simulink model "simulator_prototype_v2"  (R2021b)
settings: Solver=VariableStepAuto  StartTime=0.0  StopTime=60  FixedStep=0.0001  RelTol=1e-4
values from neighbouring files (symbols this model uses):
  N = length(mass)    [inertia_matrix.m]
undefined symbols (not defined in the file or in its folder): X, Y, Z
libraries: sm_lib x47, nesl_utility x7
(part 4 of 12)

== matlab function simulator_prototype_v2/Dynamic Model/Coriolis_vector_v2 ==
  data: dq1 input; tau_c output; dq2 input; dq3 input; dq4 input; dq5 input; dq6 input; q1 input; q2 input; q3 input; q4 input; q5 input; q6 input
function tau_c = Coriolis_vector_v2(dq1,dq2,dq3,dq4,dq5,dq6,q1,q2,q3,q4,q5,q6)
%#codegen

%    This function was generated by the Symbolic Math Toolbox version 9.0.
%    06-Nov-2021 23:01:03

t2 = conj(dq1);
t3 = conj(dq2);
t4 = conj(dq3);
t5 = conj(dq4);
t6 = conj(dq5);
t7 = conj(dq6);
t8 = conj(q1);
t9 = conj(q2);
t10 = conj(q3);
t11 = conj(q4);
t12 = conj(q5);
t13 = conj(q6);
t14 = cos(q1);
t15 = cos(q2);
t16 = cos(q4);
t17 = cos(q5);
t18 = cos(q6);
t19 = sin(q1);
t20 = sin(q2);
t21 = sin(q4);
t22 = sin(q5);
t23 = sin(q6);
t29 = q1+q2;
t50 = 9.007199254740992e+15;
t24 = cos(t8);
t25 = cos(t9);
t26 = cos(t11);
t27 = cos(t12);
t28 = cos(t13);
t30 = sin(t8);
t31 = sin(t9);
t32 = sin(t11);
t33 = sin(t12);
t34 = sin(t13);
t35 = cos(t29);
t36 = sin(t29);
t37 = t8+t9;
t51 = t17.*3.347317932164228e+33;
t52 = t22.*3.347317932164228e+33;
t56 = t14.*4.990478e-2;
t58 = t19.*4.990478e-2;
t59 = t14.*2.167433e-2;
t60 = t19.*2.167433e-2;
t61 = t16.*t18.*3.315051378778914e+33;
t62 = t14.*t15.*3.641522e-2;
t63 = t16.*t23.*3.315051378778914e+33;
t64 = t18.*t21.*3.315051378778914e+33;
t65 = t16.*t22.*1.990083581481952e+33;
t66 = t17.*t21.*1.990083581481952e+33;
t67 = t14.*t20.*3.641522e-2;
t68 = t15.*t19.*3.641522e-2;
t69 = t21.*t22.*1.990083581481952e+33;
t70 = t19.*t20.*3.641522e-2;
t74 = t19.*t20.*2.462267e-2;
t78 = t17.*t18.*5.575912001630188e+33;
t79 = t16.*t18.*6.099194893302011e+33;
t80 = t17.*t18.*1.025883768304404e+34;
t81 = t17.*t23.*5.575912001630188e+33;
t82 = t16.*t23.*6.099194893302011e+33;
t83 = t17.*t23.*1.025883768304404e+34;
t84 = t18.*t22.*1.025883768304404e+34;
t85 = t22.*t23.*5.575912001630188e+33;
t87 = t21.*t23.*6.099194893302011e+33;
t89 = t14.*t15.*2.462267e-2;
t90 = t14.*t20.*2.462267e-2;
t91 = t15.*t19.*2.462267e-2;
t93 = t21.*t22.*t23.*3.315051378778914e+33;
t105 = t17.*t21.*t23.*3.315051378778914e+33;
t116 = t17.*t18.*t21.*6.099194893302011e+33;
t118 = t18.*t21.*t22.*6.099194893302011e+33;
t127 = t21.*t22.*t23.*-6.099194893302011e+33;
t142 = t16.*7.746286054220548e+49;
t143 = t21.*7.746286054220548e+49;
t144 = t16.*t22.*1.830618490855195e+48;
t145 = t17.*t21.*1.830618490855195e+48;
t150 = t16.*t17.*1.830618490855195e+48;
t153 = t16.*t17.*7.290917220067534e+49;
t154 = t16.*t22.*7.290917220067534e+49;
t155 = t21.*t22.*7.290917220067534e+49;
t158 = t16.*6.997781708721691e+52;
t159 = t21.*6.997781708721691e+52;
t166 = t16.*t17.*t18.*5.84291401185902e+49;
t168 = t16.*t17.*t23.*5.84291401185902e+49;
t170 = t16.*t22.*t23.*5.84291401185902e+49;
t171 = t17.*t21.*t23.*5.84291401185902e+49;
t174 = t16.*t22.*7.183572847808854e+52;
t175 = t17.*t21.*7.183572847808854e+52;
t177 = t21.*t22.*7.183572847808854e+52;
t178 = t16.*t17.*t18.*1.075008113939401e+50;
t179 = t16.*t17.*t23.*1.075008113939401e+50;
t180 = t16.*t18.*t22.*1.075008113939401e+50;
t181 = t17.*t18.*t21.*1.075008113939401e+50;
t183 = (q3.*t50)./9.007199254740992e+15;
t184 = t16.*t18.*1.196628789628727e+53;
t185 = t16.*t23.*1.196628789628727e+53;
t186 = t18.*t21.*1.196628789628727e+53;
t187 = (t10.*t50)./9.007199254740992e+15;
t191 = t16.*t18.*2.201616617347892e+53;
t192 = t16.*t23.*2.201616617347892e+53;
t193 = q3.*t50.*2.220446049250313e-16i;
t194 = t21.*t23.*2.201616617347892e+53;
t199 = t10.*t50.*2.220446049250313e-16i;
t206 = q3.*t50.*1.110223024625157e-16i;
t210 = t17.*t21.*t23.*1.196628789628727e+53;
t212 = t21.*t22.*t23.*1.196628789628727e+53;
t214 = t10.*t50.*1.110223024625157e-16i;
t219 = t17.*t18.*t21.*2.201616617347892e+53;
t221 = t18.*t21.*t22.*2.201616617347892e+53;
t232 = t16.*t17.*t50.*4.323455642275676e+17i;
t233 = t16.*t22.*t50.*4.323455642275676e+17i;
t234 = t21.*t22.*t50.*4.323455642275676e+17i;
t242 = t21.*t22.*t23.*-2.201616617347892e+53;
t247 = t16.*t18.*t50.*7.201947557068188e+17i;
t248 = t16.*t23.*t50.*1.325049802940888e+18i;
t249 = t18.*t21.*t50.*1.325049802940888e+18i;
t251 = t18.*t21.*t50.*7.201947557068188e+17i;
t253 = t21.*t23.*t50.*1.325049802940888e+18i;
t254 = t21.*t23.*t50.*7.201947557068188e+17i;
t278 = t16.*t17.*t18.*t50.*1.325049802940888e+18i;
t282 = t16.*t18.*t22.*t50.*1.325049802940888e+18i;
t284 = t16.*t17.*t23.*t50.*7.201947557068188e+17i;
t289 = t16.*t22.*t23.*t50.*7.201947557068188e+17i;
t297 = t16.*t22.*t23.*t50.*-1.325049802940888e+18i;
t298 = t18.*t21.*t22.*t50.*-1.325049802940888e+18i;
t299 = t21.*t22.*t23.*t50.*-7.201947557068188e+17i;
t353 = t17.*t50.*1.746965228796509e+32i;
t355 = t22.*t50.*1.746965228796509e+32i;
t375 = t16.*t50.*4.394953650240249e+33i;
t377 = t21.*t50.*4.394953650240249e+33i;
t379 = t17.*t21.*t50.*1.03862462117543e+32i;
t383 = t21.*t22.*t50.*1.03862462117543e+32i;
t385 = t17.*t50.*6.957746211523004e+33i;
t386 = t22.*t50.*6.957746211523004e+33i;
t390 = t16.*t17.*t50.*1.03862462117543e+32i;
t394 = t16.*t22.*t50.*4.136594366080324e+33i;
t395 = t17.*t21.*t50.*4.136594366080324e+33i;
t396 = t21.*t22.*t50.*4.136594366080324e+33i;
t399 = t16.*t50.*3.97028021545552e+36i;
t400 = t21.*t50.*3.97028021545552e+36i;
t401 = t17.*t18.*t50.*1.025883768304404e+34i;
t402 = t17.*t23.*t50.*5.575912001630188e+33i;
t403 = t18.*t22.*t50.*5.575912001630188e+33i;
t404 = t18.*t22.*t50.*1.025883768304404e+34i;
t406 = t22.*t23.*t50.*5.575912001630188e+33i;
t409 = t22.*t23.*t50.*1.025883768304404e+34i;
t415 = t16.*t17.*t23.*t50.*3.315051378778914e+33i;
t416 = t17.*t18.*t21.*t50.*3.315051378778914e+33i;
t417 = t17.*t21.*t23.*t50.*3.315051378778914e+33i;
t418 = t21.*t22.*t23.*t50.*3.315051378778914e+33i;
t433 = t16.*t17.*t50.*4.075691174875038e+36i;
t435 = t16.*t22.*t50.*4.075691174875038e+36i;
t436 = t21.*t22.*t50.*4.075691174875038e+36i;
t440 = t16.*t17.*t18.*t50.*6.099194893302011e+33i;
t443 = t17.*t18.*t21.*t50.*6.099194893302011e+33i;
t446 = t17.*t21.*t23.*t50.*6.099194893302011e+33i;
t447 = t18.*t21.*t22.*t50.*6.099194893302011e+33i;
t448 = t16.*t18.*t50.*6.789225223739216e+36i;
t449 = t16.*t23.*t50.*1.249115114148252e+37i;
t450 = t18.*t21.*t50.*1.249115114148252e+37i;
t451 = t18.*t21.*t50.*6.789225223739216e+36i;
t453 = t21.*t23.*t50.*1.249115114148252e+37i;
t454 = t21.*t23.*t50.*6.789225223739216e+36i;
t472 = t16.*t17.*t18.*t50.*1.249115114148252e+37i;
t476 = t16.*t18.*t22.*t50.*1.249115114148252e+37i;
t477 = t16.*t17.*t23.*t50.*6.789225223739216e+36i;
t483 = t16.*t22.*t23.*t50.*6.789225223739216e+36i;
t494 = t16.*t22.*t23.*t50.*-1.249115114148252e+37i;
t495 = t18.*t21.*t22.*t50.*-1.249115114148252e+37i;
t496 = t21.*t22.*t23.*t50.*-6.789225223739216e+36i;
t583 = t14.*t15.*3.15365435562893e-2;
t584 = t14.*t20.*3.15365435562893e-2;
t585 = t15.*t19.*3.15365435562893e-2;
t586 = t14.*t15.*2.561099610858757e-2;
t588 = t19.*t20.*3.15365435562893e-2;
t589 = t14.*t20.*2.561099610858757e-2;
t590 = t15.*t19.*2.561099610858757e-2;
t592 = t19.*t20.*2.561099610858757e-2;
t597 = t14.*t15.*1.57299335562893e-2;
t600 = t14.*t20.*1.57299335562893e-2;
t601 = t15.*t19.*1.57299335562893e-2;
t603 = t19.*t20.*1.57299335562893e-2;
t604 = t14.*t15.*4.804434610858757e-2;
t605 = t14.*t20.*4.804434610858757e-2;
t606 = t15.*t19.*4.804434610858757e-2;
t607 = t19.*t20.*4.804434610858757e-2;
t626 = t14.*t15.*1.919581841189621e-2;
t628 = t14.*t15.*4.735389991350965e-2;
t632 = t14.*t20.*1.919581841189621e-2;
t633 = t15.*t19.*1.919581841189621e-2;
t635 = t14.*t20.*4.735389991350965e-2;
t636 = t15.*t19.*4.735389991350965e-2;
t638 = t19.*t20.*1.919581841189621e-2;
t639 = t19.*t20.*4.735389991350965e-2;
t640 = t14.*t15.*2.273122991350965e-2;
t641 = t14.*t15.*3.603517512464e-2;
t642 = t14.*t20.*2.273122991350965e-2;
t643 = t15.*t19.*2.273122991350965e-2;
t645 = t14.*t20.*3.603517512464e-2;
t646 = t15.*t19.*3.603517512464e-2;
t647 = t19.*t20.*2.273122991350965e-2;
t649 = t19.*t20.*3.603517512464e-2;
t653 = t14.*t15.*1.141250512464e-2;
t654 = t14.*t20.*1.141250512464e-2;
t655 = t15.*t19.*1.141250512464e-2;
t656 = t19.*t20.*1.141250512464e-2;
t661 = t14.*t15.*5.561103841189621e-2;
t663 = t14.*t20.*5.561103841189621e-2;
t664 = t15.*t19.*5.561103841189621e-2;
t666 = t19.*t20.*5.561103841189621e-2;
t667 = t14.*t15.*3.823389842399381e-2;
t668 = t14.*t20.*3.823389842399381e-2;
t669 = t15.*t19.*3.823389842399381e-2;
t671 = t14.*t15.*7.464911842399381e-2;
t674 = t19.*t20.*3.823389842399381e-2;
t675 = t14.*t20.*7.464911842399381e-2;
t676 = t15.*t19.*7.464911842399381e-2;
t679 = t19.*t20.*7.464911842399381e-2;
t703 = t14.*t15.*t16.*t22.*2.498039274760989e-3;
t704 = t14.*t16.*t17.*t20.*2.498039274760989e-3;
t705 = t15.*t16.*t17.*t19.*2.498039274760989e-3;
t706 = t14.*t15.*t21.*t22.*2.498039274760989e-3;
t707 = t14.*t16.*t20.*t22.*2.498039274760989e-3;
t708 = t15.*t16.*t19.*t22.*2.498039274760989e-3;
t709 = t16.*t17.*t19.*t20.*2.498039274760989e-3;
t711 = t14.*t15.*t16.*t17.*5.478347731418506e-3;
t712 = t14.*t20.*t21.*t22.*2.498039274760989e-3;
t713 = t15.*t19.*t21.*t22.*2.498039274760989e-3;
t714 = t16.*t19.*t20.*t22.*2.498039274760989e-3;
t719 = t14.*t15.*t16.*t22.*5.478347731418506e-3;
t720 = t14.*t15.*t17.*t21.*5.478347731418506e-3;
t721 = t14.*t16.*t17.*t20.*5.478347731418506e-3;
t722 = t15.*t16.*t17.*t19.*5.478347731418506e-3;
t723 = t19.*t20.*t21.*t22.*2.498039274760989e-3;
t726 = t14.*t16.*t20.*t22.*5.478347731418506e-3;
t727 = t14.*t17.*t20.*t21.*5.478347731418506e-3;
t728 = t15.*t16.*t19.*t22.*5.478347731418506e-3;
t729 = t15.*t17.*t19.*t21.*5.478347731418506e-3;
t730 = t16.*t17.*t19.*t20.*5.478347731418506e-3;
t731 = t16.*t19.*t20.*t22.*5.478347731418506e-3;
t732 = t17.*t19.*t20.*t21.*5.478347731418506e-3;
t742 = t14.*t15.*t16.*t17.*2.498039274760989e-3;
t748 = t14.*t15.*t16.*t17.*4.201698731382561e-3;
t749 = t14.*t15.*t16.*t22.*4.201698731382561e-3;
t750 = t14.*t16.*t17.*t20.*4.201698731382561e-3;
t751 = t15.*t16.*t17.*t19.*4.201698731382561e-3;
t752 = t14.*t15.*t21.*t22.*4.201698731382561e-3;
t753 = t14.*t16.*t20.*t22.*4.201698731382561e-3;
t754 = t15.*t16.*t19.*t22.*4.201698731382561e-3;
t755 = t16.*t17.*t19.*t20.*4.201698731382561e-3;
t760 = t14.*t20.*t21.*t22.*4.201698731382561e-3;
t761 = t15.*t19.*t21.*t22.*4.201698731382561e-3;
t762 = t16.*t19.*t20.*t22.*4.201698731382561e-3;
t766 = t19.*t20.*t21.*t22.*4.201698731382561e-3;
t768 = t14.*t15.*t16.*t17.*9.214573584066668e-3;
t769 = t14.*t15.*t16.*t22.*9.214573584066668e-3;
t770 = t14.*t15.*t17.*t21.*9.214573584066668e-3;
t771 = t14.*t16.*t17.*t20.*9.214573584066668e-3;
t772 = t15.*t16.*t17.*t19.*9.214573584066668e-3;
t773 = t14.*t16.*t20.*t22.*9.214573584066668e-3;
t774 = t14.*t17.*t20.*t21.*9.214573584066668e-3;
t775 = t15.*t16.*t19.*t22.*9.214573584066668e-3;
t776 = t15.*t17.*t19.*t21.*9.214573584066668e-3;
t777 = t16.*t17.*t19.*t20.*9.214573584066668e-3;
t778 = t16.*t19.*t20.*t22.*9.214573584066668e-3;
t779 = t17.*t19.*t20.*t21.*9.214573584066668e-3;
t780 = t19.*t20.*t21.*2.842045365580232e-6;
t788 = t14.*t15.*t16.*2.538961213904336e-3;
t789 = t14.*t15.*t21.*2.538961213904336e-3;
t790 = t14.*t16.*t20.*2.538961213904336e-3;
t791 = t15.*t16.*t19.*2.538961213904336e-3;
t792 = t14.*t20.*t21.*2.538961213904336e-3;
t793 = t15.*t19.*t21.*2.538961213904336e-3;
t794 = t16.*t19.*t20.*2.538961213904336e-3;
t795 = t19.*t20.*t21.*2.538961213904336e-3;
t798 = t14.*t15.*t16.*2.842045365580232e-6;
t800 = t14.*t15.*t21.*2.842045365580232e-6;
t801 = t14.*t16.*t20.*2.842045365580232e-6;
t802 = t15.*t16.*t19.*2.842045365580232e-6;
t803 = t14.*t20.*t21.*2.842045365580232e-6;
t804 = t15.*t19.*t21.*2.842045365580232e-6;
t805 = t16.*t19.*t20.*2.842045365580232e-6;
t806 = t14.*t20.*t21.*4.780316517734772e-6;
t807 = t15.*t19.*t21.*4.780316517734772e-6;
t808 = t16.*t19.*t20.*4.780316517734772e-6;
t810 = t19.*t20.*t21.*4.780316517734772e-6;
t811 = t14.*t15.*t16.*4.270529378491088e-3;
t813 = t14.*t15.*t21.*4.270529378491088e-3;
t814 = t14.*t16.*t20.*4.270529378491088e-3;
t815 = t15.*t16.*t19.*4.270529378491088e-3;
t816 = t14.*t20.*t21.*4.270529378491088e-3;
t817 = t15.*t19.*t21.*4.270529378491088e-3;
t818 = t16.*t19.*t20.*4.270529378491088e-3;
t819 = t19.*t20.*t21.*4.270529378491088e-3;
t821 = t14.*t15.*t16.*4.780316517734772e-6;
t822 = t14.*t15.*t21.*4.780316517734772e-6;
t823 = t14.*t16.*t20.*4.780316517734772e-6;
t824 = t15.*t16.*t19.*4.780316517734772e-6;
t38 = cos(t37);
t39 = sin(t37);
t40 = t36.*7.742227997977903e+15;
t41 = t35.*4.602992943936994e+15;
t42 = t36.*4.602992943936994e+15;
t43 = t35.*7.742227997977903e+15;
t53 = t27.*3.347317932164228e+33;
t54 = t33.*3.347317932164228e+33;
t55 = t35.*1.580661e-2;
t57 = t36.*1.580661e-2;
t73 = -t60;
t75 = -t61;
t76 = -t62;
t77 = -t66;
t86 = t35.*2.243335e-2;
t88 = t36.*2.243335e-2;
t92 = -t74;
t94 = -t83;
t96 = -t87;
t98 = t26.*t28.*3.315051378778914e+33;
t99 = t26.*t34.*3.315051378778914e+33;
t100 = t28.*t32.*3.315051378778914e+33;
t101 = t26.*t33.*1.990083581481952e+33;
t102 = t27.*t32.*1.990083581481952e+33;
t103 = t32.*t33.*1.990083581481952e+33;
t104 = t22.*t63;
t106 = t22.*t64;
t107 = t27.*t28.*5.575912001630188e+33;
t108 = t26.*t28.*6.099194893302011e+33;
t109 = t27.*t28.*1.025883768304404e+34;
t110 = t27.*t34.*5.575912001630188e+33;
t111 = t26.*t34.*6.099194893302011e+33;
t112 = t27.*t34.*1.025883768304404e+34;
t113 = t28.*t33.*1.025883768304404e+34;
t114 = t33.*t34.*5.575912001630188e+33;
t115 = t22.*t79;
t117 = t32.*t34.*6.099194893302011e+33;
t119 = t22.*t87;
t122 = -t105;
t125 = -t116;
t129 = t27.*t32.*t34.*3.315051378778914e+33;
t132 = t32.*t33.*t34.*3.315051378778914e+33;
t135 = t27.*t28.*t32.*6.099194893302011e+33;
t136 = t28.*t32.*t33.*6.099194893302011e+33;
t139 = t32.*t33.*t34.*-6.099194893302011e+33;
t146 = t26.*7.746286054220548e+49;
t147 = t32.*7.746286054220548e+49;
t148 = -t142;
t149 = -t143;
t156 = -t154;
t157 = -t155;
t160 = t26.*t27.*1.830618490855195e+48;
t161 = t26.*t33.*1.830618490855195e+48;
t162 = t27.*t32.*1.830618490855195e+48;
t163 = t26.*t33.*7.290917220067534e+49;
t164 = t32.*t33.*7.290917220067534e+49;
t165 = -t159;
t167 = t26.*6.997781708721691e+52;
t169 = t32.*6.997781708721691e+52;
t172 = t26.*t27.*7.290917220067534e+49;
t188 = cos(t183);
t189 = sin(t183);
t190 = -t179;
t195 = t26.*t27.*t34.*5.84291401185902e+49;
t196 = t26.*t33.*t34.*5.84291401185902e+49;
t197 = t27.*t32.*t34.*5.84291401185902e+49;
t198 = -t184;
t200 = exp(t193);
t201 = cos(t187);
t202 = sin(t187);
t203 = t26.*t33.*7.183572847808854e+52;
t204 = t27.*t32.*7.183572847808854e+52;
t205 = t32.*t33.*7.183572847808854e+52;
t207 = -t194;
t208 = t26.*t27.*t28.*5.84291401185902e+49;
t209 = t22.*t185;
t211 = t22.*t186;
t213 = -t199;
t215 = exp(t206);
t216 = t26.*t28.*2.201616617347892e+53;
t217 = t26.*t34.*2.201616617347892e+53;
t218 = t22.*t191;
t220 = t32.*t34.*2.201616617347892e+53;
t222 = t22.*t194;
t223 = t26.*t27.*t28.*1.075008113939401e+50;
t224 = t26.*t28.*1.196628789628727e+53;
t225 = t26.*t27.*t34.*1.075008113939401e+50;
t226 = t26.*t28.*t33.*1.075008113939401e+50;
t227 = t27.*t28.*t32.*1.075008113939401e+50;
t228 = -t206;
t230 = t26.*t34.*1.196628789628727e+53;
t231 = t28.*t32.*1.196628789628727e+53;
t235 = -t214;
t241 = exp(t214);
t245 = -t232;
t246 = -t234;
t255 = t26.*t33.*t50.*4.323455642275676e+17i;
t257 = t32.*t33.*t50.*4.323455642275676e+17i;
t260 = t27.*t32.*t34.*1.196628789628727e+53;
t263 = t32.*t33.*t34.*1.196628789628727e+53;
t266 = -t248;
t267 = -t249;
t269 = -t253;
t270 = -t254;
t272 = t27.*t28.*t32.*2.201616617347892e+53;
t273 = t26.*t27.*t50.*4.323455642275676e+17i;
t274 = t28.*t32.*t33.*2.201616617347892e+53;
t276 = t32.*t33.*t34.*-2.201616617347892e+53;
t277 = t26.*t28.*t50.*7.201947557068188e+17i;
t279 = t26.*t34.*t50.*1.325049802940888e+18i;
t280 = t28.*t32.*t50.*1.325049802940888e+18i;
t281 = t28.*t32.*t50.*7.201947557068188e+17i;
t283 = t32.*t34.*t50.*1.325049802940888e+18i;
t285 = t22.*t247;
t286 = t32.*t34.*t50.*7.201947557068188e+17i;
t287 = t22.*t248;
t288 = t22.*t249;
t290 = t22.*t254;
t294 = -t278;
t296 = -t284;
t301 = t26.*t27.*t28.*t50.*1.325049802940888e+18i;
t302 = t26.*t28.*t33.*t50.*1.325049802940888e+18i;
t303 = t26.*t27.*t34.*t50.*7.201947557068188e+17i;
t307 = t26.*t33.*t34.*t50.*7.201947557068188e+17i;
t310 = t26.*t28.*t33.*t50.*-7.201947557068188e+17i;
t312 = t24.*7.234522890390001e-5;
t313 = t30.*7.234522890390001e-5;
t314 = t24.*1.665736718274e-4;
t315 = t24.*4.418500737171001e-4;
t316 = t30.*1.665736718274e-4;
t317 = t30.*4.418500737171001e-4;
t318 = t24.*1.0173523574586e-3;
t320 = t30.*1.0173523574586e-3;
t321 = t24.*1.4420704809832e-3;
t322 = t30.*1.4420704809832e-3;
t326 = t24.*5.42809301582e-4;
t327 = t30.*2.35749519977e-4;
t328 = t30.*5.42809301582e-4;
t329 = t24.*3.62675502933e-4;
t330 = t24.*6.263109763852e-4;
t331 = t30.*3.62675502933e-4;
t332 = t30.*6.263109763852e-4;
t333 = t24.*1.575149421255e-4;
t334 = t30.*1.575149421255e-4;
t338 = t24.*2.35749519977e-4;
t357 = t24.*t25.*2.64642149067e-4;
t358 = t24.*t31.*2.64642149067e-4;
t359 = t25.*t30.*2.64642149067e-4;
t360 = t30.*t31.*2.64642149067e-4;
t364 = t24.*t31.*1.789415608245e-4;
t365 = t25.*t30.*1.789415608245e-4;
t367 = t30.*t31.*1.789415608245e-4;
t368 = -t353;
t373 = t27.*t50.*1.746965228796509e+32i;
t376 = t33.*t50.*1.746965228796509e+32i;
t378 = t24.*t25.*1.789415608245e-4;
t381 = t26.*t50.*4.394953650240249e+33i;
t384 = t32.*t50.*4.394953650240249e+33i;
t388 = -t375;
t391 = -t379;
t392 = -t383;
t397 = t27.*t50.*6.957746211523004e+33i;
t398 = t33.*t50.*6.957746211523004e+33i;
t405 = t26.*t27.*t50.*1.03862462117543e+32i;
t407 = -t394;
t408 = -t395;
t411 = t27.*t32.*t50.*1.03862462117543e+32i;
t412 = t32.*t33.*t50.*1.03862462117543e+32i;
t419 = -t399;
t420 = -t400;
t421 = t26.*t33.*t50.*4.136594366080324e+33i;
t422 = t27.*t32.*t50.*4.136594366080324e+33i;
t423 = t32.*t33.*t50.*4.136594366080324e+33i;
t424 = -t401;
t425 = -t402;
t427 = -t409;
t428 = t26.*t50.*3.97028021545552e+36i;
t430 = t32.*t50.*3.97028021545552e+36i;
t431 = -t416;
t432 = -t417;
t434 = -t418;
t437 = t27.*t28.*t50.*1.025883768304404e+34i;
t438 = t27.*t34.*t50.*5.575912001630188e+33i;
t439 = t28.*t33.*t50.*5.575912001630188e+33i;
t441 = t28.*t33.*t50.*1.025883768304404e+34i;
t442 = t33.*t34.*t50.*5.575912001630188e+33i;
t444 = t33.*t34.*t50.*1.025883768304404e+34i;
t452 = -t436;
t457 = -t443;
t459 = -t447;
t460 = t26.*t33.*t50.*4.075691174875038e+36i;
t461 = t32.*t33.*t50.*4.075691174875038e+36i;
t462 = t26.*t27.*t34.*t50.*3.315051378778914e+33i;
t463 = t27.*t28.*t32.*t50.*3.315051378778914e+33i;
t464 = -t449;
t465 = -t450;
t466 = t27.*t32.*t34.*t50.*3.315051378778914e+33i;
t467 = -t453;
t468 = -t454;
t469 = t32.*t33.*t34.*t50.*3.315051378778914e+33i;
t470 = t26.*t27.*t50.*4.075691174875038e+36i;
t473 = t26.*t34.*t50.*1.249115114148252e+37i;
t474 = t28.*t32.*t50.*1.249115114148252e+37i;
tau_c = ft_1({t100,t101,t102,t103,t104,t105,t106,t107,t108,t109,t110,t111,t112,t113,t114,t115,t116,t117,t118,t119,t122,t125,t127,t129,t132,t135,t136,t139,t14,t142,t143,t144,t145,t146,t147,t148,t149,t15,t150,t153,t154,t155,t156,t157,t158,t159,t16,t160,t161,t162,t163,t164,t165,t166,t167,t168,t169,t17,t170,t171,t172,t174,t175,t177,t178,t179,t18,t180,t181,t184,t185,t186,t188,t189,t19,t190,t191,t192,t194,t195,t196,t197,t198,t2,t20,t200,t201,t202,t203,t204,t205,t207,t208,t209,t21,t210,t211,t212,t213,t215,t216,t217,t218,t219,t22,t220,t221,t222,t223,t224,t225,t226,t227,t23,t230,t231,t232,t233,t234,t235,t24,t241,t242,t245,t246,t247,t248,t249,t25,t251,t253,t254,t255,t257,t26,t260,t263,t266,t267,t269,t27,t270,t272,t273,t274,t276,t277,t278,t279,t28,t280,t281,t282,t283,t284,t285,t286,t287,t288,t289,t290,t294,t296,t297,t298,t299,t3,t30,t301,t302,t303,t307,t31,t310,t312,t313,t314,t315,t316,t317,t318,t32,t320,t321,t322,t326,t327,t328,t329,t33,t330,t331,t332,t333,t334,t338,t34,t35,t353,t355,t357,t358,t359,t36,t360,t364,t365,t367,t368,t373,t375,t376,t377,t378,t379,t38,t381,t383,t384,t385,t386,t388,t39,t390,t391,t392,t394,t395,t396,t397,t398,t399,t4,t40,t400,t401,t402,t403,t404,t405,t406,t407,t408,t409,t41,t411,t412,t415,t416,t417,t418,t419,t42,t420,t421,t422,t423,t424,t425,t427,t428,t43,t430,t431,t432,t433,t434,t435,t436,t437,t438,t439,t440,t441,t442,t443,t444,t446,t447,t448,t449,t450,t451,t452,t453,t454,t457,t459,t460,t461,t462,t463,t464,t465,t466,t467,t468,t469,t470,t472,t473,t474,t476,t477,t483,t494,t495,t496,t5,t50,t51,t52,t53,t54,t55,t56,t57,t58,t583,t584,t585,t586,t588,t589,t59,t590,t592,t597,t6,t60,t600,t601,t603,t604,t605,t606,t607,t61,t626,t628,t63,t632,t633,t635,t636,t638,t639,t64,t640,t641,t642,t643,t645,t646,t647,t649,t65,t653,t654,t655,t656,t66,t661,t663,t664,t666,t667,t668,t669,t67,t671,t674,t675,t676,t679,t68,t69,t7,t70,t703,t704,t705,t706,t707,t708,t709,t711,t712,t713,t714,t719,t720,t721,t722,t723,t726,t727,t728,t729,t73,t730,t731,t732,t742,t748,t749,t75,t750,t751,t752,t753,t754,t755,t76,t760,t761,t762,t766,t768,t769,t77,t770,t771,t772,t773,t774,t775,t776,t777,t778,t779,t78,t780,t788,t789,t79,t790,t791,t792,t793,t794,t795,t798,t80,t800,t801,t802,t803,t804,t805,t806,t807,t808,t81,t810,t811,t813,t814,t815,t816,t817,t818,t819,t82,t821,t822,t823,t824,t83,t84,t85,t86,t87,t88,t89,t90,t91,t92,t93,t94,t96,t98,t99});
end
function tau_c = ft_1(ct)
t100 = ct{1};
t101 = ct{2};
t102 = ct{3};
t103 = ct{4};
t104 = ct{5};
t105 = ct{6};
t106 = ct{7};
t107 = ct{8};
t108 = ct{9};
t109 = ct{10};
t110 = ct{11};
t111 = ct{12};
t112 = ct{13};
t113 = ct{14};
t114 = ct{15};
t115 = ct{16};
t116 = ct{17};
t117 = ct{18};
t118 = ct{19};
t119 = ct{20};
t122 = ct{21};
t125 = ct{22};
t127 = ct{23};
t129 = ct{24};
t132 = ct{25};
t135 = ct{26};
t136 = ct{27};
t139 = ct{28};
t14 = ct{29};
t142 = ct{30};
t143 = ct{31};
t144 = ct{32};
t145 = ct{33};
t146 = ct{34};
t147 = ct{35};
t148 = ct{36};
t149 = ct{37};
t15 = ct{38};
t150 = ct{39};
t153 = ct{40};
t154 = ct{41};
t155 = ct{42};
t156 = ct{43};
t157 = ct{44};
t158 = ct{45};
t159 = ct{46};
t16 = ct{47};
t160 = ct{48};
t161 = ct{49};
t162 = ct{50};
t163 = ct{51};
t164 = ct{52};
t165 = ct{53};
t166 = ct{54};
t167 = ct{55};
t168 = ct{56};
t169 = ct{57};
t17 = ct{58};
t170 = ct{59};
t171 = ct{60};
t172 = ct{61};
t174 = ct{62};
t175 = ct{63};
t177 = ct{64};
t178 = ct{65};
t179 = ct{66};
t18 = ct{67};
t180 = ct{68};
t181 = ct{69};
t184 = ct{70};
t185 = ct{71};
t186 = ct{72};
t188 = ct{73};
t189 = ct{74};
t19 = ct{75};
t190 = ct{76};
t191 = ct{77};
t192 = ct{78};
t194 = ct{79};
t195 = ct{80};
t196 = ct{81};
t197 = ct{82};
t198 = ct{83};
t2 = ct{84};
t20 = ct{85};
t200 = ct{86};
t201 = ct{87};
t202 = ct{88};
t203 = ct{89};
t204 = ct{90};
t205 = ct{91};
t207 = ct{92};
t208 = ct{93};
t209 = ct{94};
t21 = ct{95};
t210 = ct{96};
t211 = ct{97};
t212 = ct{98};
t213 = ct{99};
t215 = ct{100};
t216 = ct{101};
t217 = ct{102};
t218 = ct{103};
t219 = ct{104};
t22 = ct{105};
t220 = ct{106};
t221 = ct{107};
t222 = ct{108};
t223 = ct{109};
t224 = ct{110};
t225 = ct{111};
t226 = ct{112};
t227 = ct{113};
t23 = ct{114};
t230 = ct{115};
t231 = ct{116};
t232 = ct{117};
t233 = ct{118};
t234 = ct{119};
t235 = ct{120};
t24 = ct{121};
t241 = ct{122};
t242 = ct{123};
t245 = ct{124};
t246 = ct{125};
t247 = ct{126};
t248 = ct{127};
t249 = ct{128};
t25 = ct{129};
t251 = ct{130};
t253 = ct{131};
t254 = ct{132};
t255 = ct{133};
t257 = ct{134};
t26 = ct{135};
t260 = ct{136};
t263 = ct{137};
t266 = ct{138};
t267 = ct{139};
t269 = ct{140};
t27 = ct{141};
t270 = ct{142};
t272 = ct{143};
t273 = ct{144};
t274 = ct{145};
t276 = ct{146};
t277 = ct{147};
t278 = ct{148};
t279 = ct{149};
t28 = ct{150};
t280 = ct{151};
t281 = ct{152};
t282 = ct{153};
t283 = ct{154};
t284 = ct{155};
t285 = ct{156};
t286 = ct{157};
t287 = ct{158};
t288 = ct{159};
t289 = ct{160};
t290 = ct{161};
t294 = ct{162};
t296 = ct{163};
t297 = ct{164};
t298 = ct{165};
t299 = ct{166};
t3 = ct{167};
t30 = ct{168};
t301 = ct{169};
t302 = ct{170};
t303 = ct{171};
t307 = ct{172};
t31 = ct{173};
t310 = ct{174};
t312 = ct{175};
t313 = ct{176};
t314 = ct{177};
t315 = ct{178};
t316 = ct{179};
t317 = ct{180};
t318 = ct{181};
t32 = ct{182};
t320 = ct{183};
t321 = ct{184};
t322 = ct{185};
t326 = ct{186};
t327 = ct{187};
t328 = ct{188};
t329 = ct{189};
t33 = ct{190};
t330 = ct{191};
t331 = ct{192};
t332 = ct{193};
t333 = ct{194};
t334 = ct{195};
t338 = ct{196};
t34 = ct{197};
t35 = ct{198};
t353 = ct{199};
t355 = ct{200};
t357 = ct{201};
t358 = ct{202};
t359 = ct{203};
t36 = ct{204};
t360 = ct{205};
t364 = ct{206};
t365 = ct{207};
t367 = ct{208};
t368 = ct{209};
t373 = ct{210};
t375 = ct{211};
t376 = ct{212};
t377 = ct{213};
t378 = ct{214};
t379 = ct{215};
t38 = ct{216};
t381 = ct{217};
t383 = ct{218};
t384 = ct{219};
t385 = ct{220};
t386 = ct{221};
t388 = ct{222};
t39 = ct{223};
t390 = ct{224};
t391 = ct{225};
t392 = ct{226};
t394 = ct{227};
t395 = ct{228};
t396 = ct{229};
t397 = ct{230};
t398 = ct{231};
t399 = ct{232};
t4 = ct{233};
t40 = ct{234};
t400 = ct{235};
t401 = ct{236};
t402 = ct{237};
t403 = ct{238};
t404 = ct{239};
t405 = ct{240};
t406 = ct{241};
t407 = ct{242};
t408 = ct{243};
t409 = ct{244};
t41 = ct{245};
t411 = ct{246};
t412 = ct{247};
t415 = ct{248};
t416 = ct{249};
t417 = ct{250};
t418 = ct{251};
t419 = ct{252};
t42 = ct{253};
t420 = ct{254};
t421 = ct{255};
t422 = ct{256};
t423 = ct{257};
t424 = ct{258};
t425 = ct{259};
t427 = ct{260};
t428 = ct{261};
t43 = ct{262};
t430 = ct{263};
t431 = ct{264};
t432 = ct{265};
t433 = ct{266};
t434 = ct{267};
t435 = ct{268};
t436 = ct{269};
t437 = ct{270};
t438 = ct{271};
t439 = ct{272};
t440 = ct{273};
t441 = ct{274};
t442 = ct{275};
t443 = ct{276};
t444 = ct{277};
t446 = ct{278};
t447 = ct{279};
t448 = ct{280};
t449 = ct{281};
t450 = ct{282};
t451 = ct{283};
t452 = ct{284};
t453 = ct{285};
t454 = ct{286};
t457 = ct{287};
t459 = ct{288};
t460 = ct{289};
t461 = ct{290};
t462 = ct{291};
t463 = ct{292};
t464 = ct{293};
t465 = ct{294};
t466 = ct{295};
t467 = ct{296};
t468 = ct{297};
t469 = ct{298};
t470 = ct{299};
t472 = ct{300};
t473 = ct{301};
t474 = ct{302};
t476 = ct{303};
t477 = ct{304};
t483 = ct{305};
t494 = ct{306};
t495 = ct{307};
t496 = ct{308};
t5 = ct{309};
t50 = ct{310};
t51 = ct{311};
t52 = ct{312};
t53 = ct{313};
t54 = ct{314};
t55 = ct{315};
t56 = ct{316};
t57 = ct{317};
t58 = ct{318};
t583 = ct{319};
t584 = ct{320};
t585 = ct{321};
t586 = ct{322};
t588 = ct{323};
t589 = ct{324};
t59 = ct{325};
t590 = ct{326};
t592 = ct{327};
t597 = ct{328};
t6 = ct{329};
t60 = ct{330};
t600 = ct{331};
t601 = ct{332};
t603 = ct{333};
t604 = ct{334};
t605 = ct{335};
t606 = ct{336};
t607 = ct{337};
t61 = ct{338};
t626 = ct{339};
t628 = ct{340};
t63 = ct{341};
t632 = ct{342};
t633 = ct{343};
t635 = ct{344};
t636 = ct{345};
t638 = ct{346};
t639 = ct{347};
t64 = ct{348};
t640 = ct{349};
t641 = ct{350};
t642 = ct{351};
t643 = ct{352};
t645 = ct{353};
t646 = ct{354};
t647 = ct{355};
t649 = ct{356};
t65 = ct{357};
t653 = ct{358};
t654 = ct{359};
t655 = ct{360};
t656 = ct{361};
t66 = ct{362};
t661 = ct{363};
t663 = ct{364};
t664 = ct{365};
t666 = ct{366};
t667 = ct{367};
t668 = ct{368};
t669 = ct{369};
t67 = ct{370};
t671 = ct{371};
t674 = ct{372};
t675 = ct{373};
t676 = ct{374};
t679 = ct{375};
t68 = ct{376};
t69 = ct{377};
t7 = ct{378};
t70 = ct{379};
t703 = ct{380};
t704 = ct{381};
t705 = ct{382};
t706 = ct{383};
t707 = ct{384};
t708 = ct{385};
t709 = ct{386};
t711 = ct{387};
t712 = ct{388};
t713 = ct{389};
t714 = ct{390};
t719 = ct{391};
t720 = ct{392};
t721 = ct{393};
t722 = ct{394};
t723 = ct{395};
t726 = ct{396};
t727 = ct{397};
t728 = ct{398};
t729 = ct{399};
t73 = ct{400};
t730 = ct{401};
t731 = ct{402};
t732 = ct{403};
t742 = ct{404};
t748 = ct{405};
t749 = ct{406};
t75 = ct{407};
t750 = ct{408};
t751 = ct{409};
t752 = ct{410};
t753 = ct{411};
t754 = ct{412};
t755 = ct{413};
t76 = ct{414};
t760 = ct{415};
t761 = ct{416};
t762 = ct{417};
t766 = ct{418};
t768 = ct{419};
t769 = ct{420};
t77 = ct{421};
t770 = ct{422};
t771 = ct{423};
t772 = ct{424};
t773 = ct{425};
t774 = ct{426};
t775 = ct{427};
t776 = ct{428};
t777 = ct{429};
t778 = ct{430};
t779 = ct{431};
t78 = ct{432};
t780 = ct{433};
t788 = ct{434};
t789 = ct{435};
t79 = ct{436};
t790 = ct{437};
t791 = ct{438};
t792 = ct{439};
t793 = ct{440};
t794 = ct{441};
t795 = ct{442};
t798 = ct{443};
t80 = ct{444};
t800 = ct{445};
t801 = ct{446};
t802 = ct{447};
t803 = ct{448};
t804 = ct{449};
t805 = ct{450};
t806 = ct{451};
t807 = ct{452};
t808 = ct{453};
t81 = ct{454};
t810 = ct{455};
t811 = ct{456};
t813 = ct{457};
t814 = ct{458};
t815 = ct{459};
t816 = ct{460};
t817 = ct{461};
t818 = ct{462};
t819 = ct{463};
t82 = ct{464};
t821 = ct{465};
t822 = ct{466};
t823 = ct{467};
t824 = ct{468};
t83 = ct{469};
t84 = ct{470};
t85 = ct{471};
t86 = ct{472};
t87 = ct{473};
t88 = ct{474};
t89 = ct{475};
t90 = ct{476};
t91 = ct{477};
t92 = ct{478};
t93 = ct{479};
t94 = ct{480};
t96 = ct{481};
t98 = ct{482};
t99 = ct{483};
t475 = t28.*t32.*t50.*6.789225223739216e+36i;
t478 = t22.*t448;
t479 = t32.*t34.*t50.*1.249115114148252e+37i;
t480 = t32.*t34.*t50.*6.789225223739216e+36i;
t481 = t22.*t449;
t482 = t22.*t450;
t484 = t22.*t454;
t487 = t26.*t27.*t28.*t50.*6.099194893302011e+33i;
t488 = t27.*t28.*t32.*t50.*6.099194893302011e+33i;
t489 = t27.*t32.*t34.*t50.*6.099194893302011e+33i;
t490 = t28.*t32.*t33.*t50.*6.099194893302011e+33i;
t492 = t26.*t28.*t50.*6.789225223739216e+36i;
t499 = t26.*t27.*t28.*t50.*1.249115114148252e+37i;
t500 = t26.*t28.*t33.*t50.*1.249115114148252e+37i;
t501 = t26.*t27.*t34.*t50.*6.789225223739216e+36i;
t505 = t26.*t33.*t34.*t50.*6.789225223739216e+36i;
t510 = t26.*t28.*t33.*t50.*-6.789225223739216e+36i;
t608 = -t586;
t609 = -t588;
t621 = -t603;
t622 = -t604;
t657 = -t626;
t659 = -t632;
t660 = -t633;
t665 = -t639;
t670 = -t641;
t672 = -t642;
t673 = -t643;
t677 = -t647;
t678 = -t649;
t681 = -t653;
t682 = t24.*t25.*2.273122991350965e-2;
t683 = -t661;
t684 = t24.*t31.*2.273122991350965e-2;
t685 = t25.*t30.*2.273122991350965e-2;
t686 = -t663;
t687 = -t664;
t688 = t30.*t31.*2.273122991350965e-2;
t689 = -t671;
t690 = t24.*t25.*1.141250512464e-2;
t691 = -t674;
t692 = t24.*t31.*1.141250512464e-2;
t693 = t25.*t30.*1.141250512464e-2;
t694 = t30.*t31.*1.141250512464e-2;
t695 = t24.*t25.*1.919581841189621e-2;
t699 = t24.*t31.*1.919581841189621e-2;
t700 = t25.*t30.*1.919581841189621e-2;
t702 = t30.*t31.*1.919581841189621e-2;
t710 = t24.*t25.*3.823389842399381e-2;
t715 = t24.*t31.*3.823389842399381e-2;
t716 = t25.*t30.*3.823389842399381e-2;
t724 = t30.*t31.*3.823389842399381e-2;
t743 = -t703;
t744 = -t706;
t745 = -t707;
t746 = -t708;
t747 = -t709;
t757 = -t727;
t758 = -t729;
t759 = -t730;
t763 = -t731;
t764 = -t732;
t781 = -t748;
t782 = -t752;
t783 = -t753;
t784 = -t754;
t785 = -t760;
t786 = -t761;
t787 = -t762;
t796 = -t768;
t797 = -t769;
t799 = -t779;
t809 = -t780;
t812 = -t788;
t820 = -t795;
t825 = -t803;
t826 = -t804;
t827 = -t805;
t828 = -t810;
t829 = -t811;
t830 = -t813;
t831 = -t814;
t832 = -t815;
t833 = -t821;
t1089 = t30.*t31.*5.250384412218911e-5;
t1101 = t24.*t25.*8.548515114112684e-5;
t1104 = t24.*t31.*8.548515114112684e-5;
t1105 = t25.*t30.*8.548515114112684e-5;
t1108 = t24.*t25.*1.052636211784891e-4;
t1110 = t30.*t31.*8.548515114112684e-5;
t1113 = t24.*t31.*1.052636211784891e-4;
t1114 = t25.*t30.*1.052636211784891e-4;
t1115 = t30.*t31.*1.052636211784891e-4;
t1121 = t24.*t25.*5.250384412218911e-5;
t1123 = t24.*t31.*5.250384412218911e-5;
t1124 = t25.*t30.*5.250384412218911e-5;
t1155 = t24.*t25.*1.603638597716268e-4;
t1158 = t24.*t31.*1.603638597716268e-4;
t1159 = t25.*t30.*1.603638597716268e-4;
t1162 = t30.*t31.*1.603638597716268e-4;
t1190 = t24.*t25.*1.041288275878652e-3;
t1193 = t24.*t31.*1.041288275878652e-3;
t1194 = t25.*t30.*1.041288275878652e-3;
t1196 = t30.*t31.*1.041288275878652e-3;
t1205 = t24.*t25.*5.150636339692531e-4;
t1207 = t24.*t31.*5.150636339692531e-4;
t1208 = t25.*t30.*5.150636339692531e-4;
t1210 = t30.*t31.*5.150636339692531e-4;
t1215 = t24.*t25.*8.119509961859382e-4;
t1216 = t24.*t25.*1.606961034807054e-3;
t1217 = t24.*t31.*8.119509961859382e-4;
t1218 = t25.*t30.*8.119509961859382e-4;
t1219 = t24.*t31.*1.606961034807054e-3;
t1220 = t25.*t30.*1.606961034807054e-3;
t1221 = t30.*t31.*8.119509961859382e-4;
t1222 = t30.*t31.*1.606961034807054e-3;
t1284 = t24.*t25.*t26.*2.761602722751607e-5;
t1285 = t24.*t25.*t32.*2.761602722751607e-5;
t1286 = t24.*t26.*t31.*2.761602722751607e-5;
t1287 = t25.*t26.*t30.*2.761602722751607e-5;
t1288 = t24.*t31.*t32.*2.761602722751607e-5;
t1289 = t25.*t30.*t32.*2.761602722751607e-5;
t1290 = t26.*t30.*t31.*2.761602722751607e-5;
t1293 = t30.*t31.*t32.*2.761602722751607e-5;
t1299 = t24.*t25.*t26.*t27.*5.958744043986595e-5;
t1300 = t24.*t25.*t26.*t33.*5.958744043986595e-5;
t1301 = t24.*t25.*t27.*t32.*5.958744043986595e-5;
t1302 = t24.*t26.*t27.*t31.*5.958744043986595e-5;
t1303 = t25.*t26.*t27.*t30.*5.958744043986595e-5;
t1305 = t24.*t26.*t31.*t33.*5.958744043986595e-5;
t1306 = t24.*t27.*t31.*t32.*5.958744043986595e-5;
t1307 = t25.*t26.*t30.*t33.*5.958744043986595e-5;
t1308 = t25.*t27.*t30.*t32.*5.958744043986595e-5;
t1309 = t26.*t27.*t30.*t31.*5.958744043986595e-5;
t1311 = t24.*t25.*t26.*t27.*2.71709233876478e-5;
t1312 = t26.*t30.*t31.*t33.*5.958744043986595e-5;
t1313 = t27.*t30.*t31.*t32.*5.958744043986595e-5;
t1315 = t24.*t25.*t26.*t33.*2.71709233876478e-5;
t1316 = t24.*t26.*t27.*t31.*2.71709233876478e-5;
t1317 = t25.*t26.*t27.*t30.*2.71709233876478e-5;
t1318 = t24.*t25.*t32.*t33.*2.71709233876478e-5;
t1319 = t24.*t26.*t31.*t33.*2.71709233876478e-5;
t1320 = t25.*t26.*t30.*t33.*2.71709233876478e-5;
t1321 = t26.*t27.*t30.*t31.*2.71709233876478e-5;
t1322 = t24.*t31.*t32.*t33.*2.71709233876478e-5;
t1323 = t25.*t30.*t32.*t33.*2.71709233876478e-5;
t1324 = t26.*t30.*t31.*t33.*2.71709233876478e-5;
t1328 = t30.*t31.*t32.*t33.*2.71709233876478e-5;
t1333 = t24.*t25.*t26.*t27.*4.570145693137498e-5;
t1336 = t24.*t25.*t26.*t33.*4.570145693137498e-5;
t1337 = t24.*t26.*t27.*t31.*4.570145693137498e-5;
t1338 = t25.*t26.*t27.*t30.*4.570145693137498e-5;
t1339 = t24.*t25.*t32.*t33.*4.570145693137498e-5;
t1340 = t24.*t26.*t31.*t33.*4.570145693137498e-5;
t1341 = t25.*t26.*t30.*t33.*4.570145693137498e-5;
t1342 = t26.*t27.*t30.*t31.*4.570145693137498e-5;
t1343 = t24.*t25.*t26.*3.091264323687963e-8;
t1346 = t24.*t31.*t32.*t33.*4.570145693137498e-5;
t1347 = t25.*t30.*t32.*t33.*4.570145693137498e-5;
t1348 = t26.*t30.*t31.*t33.*4.570145693137498e-5;
t1349 = t24.*t25.*t32.*3.091264323687963e-8;
t1350 = t24.*t26.*t31.*3.091264323687963e-8;
t1351 = t25.*t26.*t30.*3.091264323687963e-8;
t1354 = t30.*t31.*t32.*t33.*4.570145693137498e-5;
t1355 = t24.*t25.*t26.*4.645012099690971e-5;
t1356 = t24.*t31.*t32.*3.091264323687963e-8;
t1357 = t25.*t30.*t32.*3.091264323687963e-8;
t1358 = t26.*t30.*t31.*3.091264323687963e-8;
t1360 = t24.*t25.*t32.*4.645012099690971e-5;
t1361 = t24.*t26.*t31.*4.645012099690971e-5;
t1362 = t25.*t26.*t30.*4.645012099690971e-5;
t1363 = t30.*t31.*t32.*3.091264323687963e-8;
t1366 = t24.*t31.*t32.*4.645012099690971e-5;
t1367 = t25.*t30.*t32.*4.645012099690971e-5;
t1368 = t26.*t30.*t31.*4.645012099690971e-5;
t1369 = t30.*t31.*t32.*4.645012099690971e-5;
t1378 = t24.*t25.*t26.*t27.*1.002259954165347e-4;
t1384 = t24.*t25.*t26.*t33.*1.002259954165347e-4;
t1385 = t24.*t25.*t27.*t32.*1.002259954165347e-4;
t1386 = t24.*t26.*t27.*t31.*1.002259954165347e-4;
t1387 = t25.*t26.*t27.*t30.*1.002259954165347e-4;
t1392 = t24.*t26.*t31.*t33.*1.002259954165347e-4;
t1393 = t24.*t27.*t31.*t32.*1.002259954165347e-4;
t1394 = t25.*t26.*t30.*t33.*1.002259954165347e-4;
t1395 = t25.*t27.*t30.*t32.*1.002259954165347e-4;
t1396 = t26.*t27.*t30.*t31.*1.002259954165347e-4;
t1399 = t26.*t30.*t31.*t33.*1.002259954165347e-4;
t1400 = t27.*t30.*t31.*t32.*1.002259954165347e-4;
t1425 = t24.*t25.*t26.*5.199502473174935e-8;
t1427 = t24.*t25.*t32.*5.199502473174935e-8;
t1428 = t24.*t26.*t31.*5.199502473174935e-8;
t1429 = t25.*t26.*t30.*5.199502473174935e-8;
t1433 = t24.*t31.*t32.*5.199502473174935e-8;
t1434 = t25.*t30.*t32.*5.199502473174935e-8;
t1435 = t26.*t30.*t31.*5.199502473174935e-8;
t1438 = t30.*t31.*t32.*5.199502473174935e-8;
t44 = -t42;
t45 = t38.*4.602992943936994e+15;
t46 = t39.*4.602992943936994e+15;
t47 = t38.*7.742227997977903e+15;
t48 = t39.*7.742227997977903e+15;
t71 = -t55;
t72 = -t57;
t95 = -t86;
t97 = -t88;
t120 = -t98;
t121 = -t102;
t123 = t40+t41;
t124 = -t112;
t126 = -t117;
t128 = t33.*t99;
t130 = t33.*t100;
t133 = -t129;
t134 = t33.*t108;
t137 = t33.*t117;
t138 = -t135;
t151 = -t146;
t152 = -t147;
t173 = -t163;
t176 = -t164;
t182 = -t169;
t229 = -t208;
t236 = 1.0./t215;
t237 = t16.*t188;
t238 = t21.*t188;
t239 = -t220;
t240 = exp(t213);
t243 = -t224;
t244 = -t201;
t250 = exp(t235);
t252 = t189.*1i;
t256 = t33.*t220;
t258 = t202.*1i;
t259 = t33.*t230;
t261 = t33.*t231;
t262 = t26.*t201;
t264 = t32.*t201;
t265 = t215-1.0;
t271 = t33.*t216;
t275 = -t255;
t293 = -t277;
t295 = -t281;
t304 = t33.*t277;
t305 = t33.*t279;
t306 = t33.*t280;
t308 = t33.*t286;
t309 = -t302;
t311 = -t307;
t319 = -t313;
t323 = -t317;
t324 = t38.*3.222314966007e-4;
t325 = t39.*3.222314966007e-4;
t339 = -t327;
t340 = t39.*1.71926916309e-4;
t341 = t38.*4.567547574683999e-4;
t342 = t39.*4.567547574683999e-4;
t343 = -t332;
t344 = t38.*1.148721671835e-4;
t345 = t39.*1.148721671835e-4;
t346 = -t334;
t348 = t38.*4.573233567645e-4;
t349 = t39.*4.573233567645e-4;
t350 = t38.*1.71926916309e-4;
t363 = t38.*2.44005304615e-4;
t366 = t39.*2.44005304615e-4;
t369 = t38.*6.48243952274e-4;
t370 = t39.*6.48243952274e-4;
t371 = -t357;
t372 = t38.*1.630310061225e-4;
t374 = t39.*1.630310061225e-4;
t382 = -t367;
t389 = -t376;
t393 = -t384;
t410 = t55+t88;
t413 = -t397;
t414 = -t398;
t426 = -t405;
t445 = -t423;
t455 = -t441;
t456 = -t442;
t458 = -t444;
t471 = -t460;
t485 = -t462;
t486 = -t463;
t491 = -t470;
t493 = -t475;
t497 = -t487;
t498 = -t492;
t502 = t33.*t492;
t503 = t33.*t473;
t504 = t33.*t474;
t506 = t33.*t480;
t507 = -t499;
t508 = -t500;
t509 = -t501;
t511 = -t505;
t514 = t17.*t188.*8.595599785252598e-1;
t515 = t200.*3.064357668490995e+34;
t516 = t22.*t188.*8.595599785252598e-1;
t519 = t51.*t200;
t520 = t52.*t200;
t521 = t27.*t201.*8.595599785252598e-1;
t522 = t33.*t201.*8.595599785252598e-1;
t528 = t17.*t188.*5.157359871151559e-3;
t529 = t61.*t200;
t531 = t63.*t200;
t532 = t64.*t200;
t533 = t65.*t200;
t534 = t66.*t200;
t537 = t69.*t200;
t541 = t87.*t200;
t545 = t16.*t18.*t200.*-3.315051378778914e+33;
t547 = t16.*t22.*t200.*7.788445287802242e+33;
t548 = t17.*t21.*t200.*-1.990083581481952e+33;
t550 = t78.*t200;
t553 = t79.*t200;
t554 = t80.*t200;
t555 = t81.*t200;
t557 = t82.*t200;
t558 = t83.*t200;
t559 = t84.*t200;
t560 = t85.*t200;
t561 = t21.*t23.*t200.*-6.099194893302011e+33;
t562 = t27.*t201.*5.157359871151559e-3;
t566 = t104.*t200;
t567 = t105.*t200;
t568 = t106.*t200;
t570 = t93.*t200;
t582 = t17.*t23.*t200.*-1.025883768304404e+34;
t591 = t17.*t21.*t23.*t200.*-3.315051378778914e+33;
t595 = t115.*t200;
t596 = t116.*t200;
t599 = t118.*t200;
t602 = t119.*t200;
t619 = t17.*t18.*t21.*t200.*-6.099194893302011e+33;
t620 = t127.*t200;
t648 = t22.*t188.*8.595599785252598e-9;
t717 = -t684;
t718 = -t685;
t725 = -t688;
t736 = -t690;
t738 = -t695;
t740 = -t699;
t741 = -t700;
t756 = -t724;
t834 = t142.*t200;
t835 = t143.*t200;
t836 = t16.*t200.*-7.746286054220548e+49;
t837 = t21.*t200.*-7.746286054220548e+49;
t838 = t150.*t200;
t839 = t144.*t200;
t840 = t145.*t200;
t841 = t153.*t200;
t842 = t154.*t200;
t843 = t155.*t200;
t844 = t16.*t22.*t200.*-7.290917220067534e+49;
t845 = t21.*t22.*t200.*-7.290917220067534e+49;
t846 = t158.*t200;
t848 = t159.*t200;
t850 = (t50.*t189)./9.007199254740992e+15;
t851 = t166.*t200;
t852 = t168.*t200;
t853 = t170.*t200;
t854 = t171.*t200;
t855 = (t50.*t202)./9.007199254740992e+15;
t857 = t21.*t200.*-6.997781708721691e+52;
t860 = t16.*t22.*t200.*7.342112502577776e+52;
t861 = t178.*t200;
t862 = t179.*t200;
t863 = t180.*t200;
t864 = t181.*t200;
t866 = t174.*t200;
t867 = t175.*t200;
t869 = t177.*t200;
t874 = t50.*t188.*1.110223024625157e-16i;
t875 = t16.*t17.*t23.*t200.*-1.075008113939401e+50;
t876 = t191.*t200;
t877 = t192.*t200;
t878 = t50.*t201.*1.110223024625157e-16i;
t879 = t194.*t200;
t880 = t184.*t200;
t882 = t185.*t200;
t883 = t186.*t200;
t887 = t21.*t50.*t189.*(-1.110223024625157e-16);
t889 = t21.*t23.*t200.*-2.201616617347892e+53;
t890 = t16.*t18.*t200.*-1.196628789628727e+53;
t896 = t200.*t218;
t897 = t200.*t219;
t898 = t200.*t221;
t899 = t200.*t222;
t900 = t200.*t209;
t901 = t200.*t210;
t902 = t200.*t211;
t903 = t200.*t212;
t904 = t32.*t50.*t202.*(-1.110223024625157e-16);
t905 = t17.*t50.*t200.*7.432538878058787e+17i;
t906 = t200.*t242;
t908 = t21.*t22.*t50.*t200.*4.418873226179514e+17i;
t909 = t200.*t232;
t910 = t200.*t233;
t913 = t200.*t234;
t919 = t200.*t247;
t920 = t200.*t248;
t921 = t200.*t249;
t922 = t200.*t251;
t923 = t200.*t253;
t924 = t200.*t254;
t929 = t16.*t22.*t50.*t200.*-4.323455642275676e+17i;
t938 = t16.*t18.*t50.*t200.*-7.201947557068188e+17i;
t939 = t18.*t21.*t50.*t200.*-7.201947557068188e+17i;
t946 = t200.*t290;
t952 = t200.*t278;
t953 = t200.*t282;
t954 = t200.*t284;
t955 = t200.*t285;
t956 = t200.*t287;
t957 = t200.*t288;
t958 = t200.*t289;
t963 = t188.*7.38843356682345e-1;
t964 = t188.*2.61156643317655e-1;
t972 = (t21.*t50.*t189)./9.007199254740992e+23;
t975 = t16.*t18.*t22.*t50.*t200.*-1.325049802940888e+18i;
t977 = t16.*t22.*t23.*t50.*t200.*-7.201947557068188e+17i;
t983 = t188.*1.738813335718512e-2;
t986 = t201.*7.38843356682345e-1;
t988 = t201.*2.61156643317655e-1;
t996 = t201.*1.738813335718512e-2;
t998 = t188.*2.982577219529057e-2;
t1000 = t188.*4.721390555247569e-2;
t1001 = t17.*t188.*1.07201054193752e-2;
t1002 = t22.*t188.*1.07201054193752e-2;
t1003 = t201.*4.721390555247569e-2;
t1006 = t17.*t188.*4.888197259476159e-3;
t1008 = t22.*t188.*4.888197259476159e-3;
t1019 = t201.*2.982577219529057e-2;
t1030 = t188.*2.673231533213558e-6;
t1035 = t33.*t201.*1.07201054193752e-2;
t1039 = t188.*2.784974330421842e-6;
t1044 = t27.*t201.*4.888197259476159e-3;
t1047 = t21.*t23.*t200.*2.386997519508773e+34;
t1049 = t17.*t188.*2.691626116753997e-4;
t1055 = t18.*t21.*t200.*1.297387533374166e+34;
t1058 = t22.*t188.*8.76751178095765e-7;
t1065 = t17.*t188.*4.899491877593981e-7;
t1066 = t16.*t18.*t22.*t200.*2.386997519508773e+34;
t1067 = t27.*t201.*2.691626116753997e-4;
t1070 = t16.*t22.*t23.*t200.*1.297387533374166e+34;
t1071 = t22.*t188.*2.062943948460623e-7;
t1080 = t200.*t353;
t1082 = t200.*t355;
t1083 = t17.*t188.*3.438239914101039e-8;
t1084 = t22.*t188.*3.438239914101039e-8;
t1092 = t200.*t375;
t1096 = t200.*t377;
t1112 = t22.*t50.*t200.*-1.746965228796509e+32i;
t1126 = -t1089;
t1137 = t21.*t50.*t200.*-4.394953650240249e+33i;
t1143 = t200.*t390;
t1145 = t200.*t379;
t1148 = t200.*t383;
t1150 = -t1101;
t1154 = -t1115;
t1157 = t200.*t385;
t1161 = t200.*t386;
t1166 = t200.*t394;
t1167 = t200.*t395;
t1168 = t200.*t396;
t1170 = t16.*t17.*t50.*t200.*-1.03862462117543e+32i;
t1176 = -t1155;
t1177 = t17.*t50.*t200.*-6.957746211523004e+33i;
t1178 = t22.*t50.*t200.*-6.957746211523004e+33i;
t1179 = t200.*t401;
t1180 = t200.*t402;
t1181 = t200.*t403;
t1182 = t200.*t404;
t1183 = t200.*t406;
t1184 = t200.*t409;
t1185 = t21.*t22.*t50.*t200.*-4.136594366080324e+33i;
t1189 = t200.*t399;
t1192 = t200.*t400;
t1197 = t18.*t22.*t50.*t200.*-5.575912001630188e+33i;
t1198 = t18.*t22.*t50.*t200.*-1.025883768304404e+34i;
t1199 = t22.*t23.*t50.*t200.*-5.575912001630188e+33i;
t1201 = t200.*t415;
t1202 = t200.*t416;
t1203 = t200.*t417;
t1204 = t200.*t418;
t1212 = -t1190;
t1214 = -t1196;
t1223 = t16.*t17.*t23.*t50.*t200.*-3.315051378778914e+33i;
t1225 = t200.*t433;
t1227 = t200.*t435;
t1229 = t200.*t436;
t1230 = -t1210;
t1231 = t200.*t440;
t1232 = t200.*t443;
t1233 = t200.*t446;
t1234 = t200.*t447;
t1235 = -t1215;
t1236 = -t1216;
tau_c = ft_2({t100,t1000,t1001,t1002,t1003,t1006,t1008,t101,t1019,t102,t103,t1030,t1035,t1039,t104,t1044,t1047,t1049,t1055,t1058,t106,t1065,t1066,t1067,t107,t1070,t1071,t108,t1080,t1083,t1084,t1089,t109,t1092,t110,t1104,t1105,t1108,t111,t1110,t1112,t1113,t1114,t1115,t112,t1121,t1123,t1124,t1126,t113,t1137,t114,t1145,t1148,t115,t1150,t1154,t1158,t1159,t1162,t1166,t1167,t117,t1170,t1176,t1177,t1178,t1179,t118,t1180,t1184,t1185,t1189,t1190,t1192,t1193,t1194,t1196,t1197,t1198,t1199,t120,t1202,t1203,t1204,t1205,t1207,t1208,t121,t1210,t1212,t1214,t1217,t1218,t1219,t122,t1220,t1221,t1222,t1223,t1229,t123,t1230,t1232,t1234,t1235,t1236,t124,t125,t126,t127,t128,t1284,t1285,t1286,t1287,t1288,t1289,t129,t1290,t1293,t1299,t130,t1300,t1301,t1302,t1303,t1305,t1306,t1307,t1308,t1309,t1311,t1312,t1313,t1315,t1316,t1317,t1318,t1319,t132,t1320,t1321,t1322,t1323,t1324,t1328,t133,t1333,t1336,t1337,t1338,t1339,t134,t1340,t1341,t1342,t1343,t1346,t1347,t1348,t1349,t135,t1350,t1351,t1354,t1355,t1356,t1357,t1358,t136,t1360,t1361,t1362,t1363,t1366,t1367,t1368,t1369,t137,t1378,t138,t1384,t1385,t1386,t1387,t139,t1392,t1393,t1394,t1395,t1396,t1399,t14,t1400,t1425,t1427,t1428,t1429,t1433,t1434,t1435,t1438,t144,t145,t146,t147,t148,t149,t15,t150,t151,t152,t153,t156,t157,t158,t16,t160,t161,t162,t163,t164,t165,t166,t167,t168,t169,t17,t170,t171,t172,t173,t174,t175,t176,t177,t178,t18,t180,t181,t182,t185,t186,t188,t189,t19,t190,t191,t192,t195,t196,t197,t198,t2,t20,t200,t201,t202,t203,t204,t205,t207,t208,t209,t21,t210,t211,t212,t216,t217,t218,t219,t22,t220,t221,t223,t224,t225,t226,t227,t229,t23,t230,t231,t233,t236,t237,t238,t239,t24,t240,t241,t242,t243,t244,t245,t246,t247,t25,t250,t251,t252,t255,t256,t257,t258,t259,t26,t260,t261,t262,t263,t264,t265,t266,t267,t269,t27,t270,t271,t272,t273,t274,t275,t276,t277,t279,t28,t280,t281,t282,t283,t285,t286,t289,t293,t294,t295,t296,t297,t298,t299,t3,t30,t301,t302,t303,t304,t305,t306,t307,t308,t309,t31,t310,t311,t312,t313,t314,t315,t316,t318,t319,t32,t320,t321,t322,t323,t324,t325,t326,t328,t329,t33,t330,t331,t332,t333,t338,t339,t34,t340,t341,t342,t343,t344,t345,t346,t348,t349,t35,t350,t355,t358,t359,t36,t360,t363,t364,t365,t366,t368,t369,t370,t371,t372,t373,t374,t376,t377,t378,t38,t381,t382,t384,t385,t386,t388,t389,t39,t390,t391,t392,t393,t396,t397,t398,t4,t403,t404,t405,t406,t407,t408,t410,t411,t412,t413,t414,t415,t419,t42,t420,t421,t422,t423,t424,t425,t426,t427,t428,t43,t430,t431,t432,t433,t434,t435,t437,t438,t439,t44,t440,t441,t442,t444,t445,t446,t448,t449,t45,t450,t451,t452,t453,t454,t455,t456,t457,t458,t459,t46,t460,t461,t462,t463,t464,t465,t466,t467,t468,t469,t47,t470,t471,t472,t473,t474,t475,t476,t477,t478,t479,t48,t480,t481,t482,t483,t484,t485,t486,t487,t488,t489,t490,t491,t492,t493,t494,t495,t496,t497,t498,t499,t5,t50,t500,t501,t502,t503,t504,t505,t506,t507,t508,t509,t51,t510,t511,t514,t515,t516,t519,t52,t520,t521,t522,t528,t53,t531,t532,t533,t537,t54,t545,t547,t548,t550,t553,t554,t555,t557,t559,t56,t560,t561,t562,t566,t568,t57,t570,t58,t582,t583,t584,t585,t589,t59,t590,t591,t592,t595,t597,t599,t6,t60,t600,t601,t605,t606,t607,t608,t609,t619,t620,t621,t622,t628,t63,t635,t636,t638,t64,t640,t641,t642,t643,t645,t646,t648,t649,t65,t654,t655,t656,t657,t659,t660,t663,t664,t665,t666,t667,t668,t669,t67,t670,t672,t673,t674,t675,t676,t677,t678,t679,t68,t681,t682,t683,t684,t685,t686,t687,t689,t69,t691,t692,t693,t694,t7,t70,t702,t704,t705,t707,t708,t71,t710,t711,t712,t713,t714,t715,t716,t717,t718,t719,t72,t720,t721,t722,t723,t724,t725,t726,t728,t73,t736,t738,t740,t741,t742,t743,t744,t745,t746,t747,t749,t75,t750,t751,t755,t756,t757,t758,t759,t76,t762,t763,t764,t766,t768,t77,t770,t771,t772,t773,t774,t775,t776,t777,t778,t78,t781,t782,t783,t784,t785,t786,t787,t789,t79,t790,t791,t792,t793,t794,t796,t797,t798,t799,t80,t800,t801,t802,t806,t807,t808,t809,t81,t812,t813,t816,t817,t818,t819,t82,t820,t821,t822,t823,t824,t825,t826,t827,t828,t829,t830,t831,t832,t833,t836,t837,t838,t839,t84,t840,t841,t844,t845,t846,t85,t850,t851,t852,t853,t854,t855,t857,t86,t860,t861,t863,t864,t866,t867,t869,t874,t875,t876,t877,t878,t882,t883,t887,t889,t89,t890,t896,t897,t898,t90,t900,t901,t902,t903,t904,t905,t906,t908,t909,t91,t913,t92,t920,t921,t923,t924,t929,t93,t938,t939,t94,t946,t95,t952,t954,t956,t957,t96,t963,t964,t97,t972,t975,t977,t98,t983,t986,t988,t99,t996,t998});
end
function tau_c = ft_2(ct)
t100 = ct{1};
t1000 = ct{2};
t1001 = ct{3};
t1002 = ct{4};
t1003 = ct{5};
t1006 = ct{6};
t1008 = ct{7};
t101 = ct{8};
t1019 = ct{9};
t102 = ct{10};
t103 = ct{11};
t1030 = ct{12};
t1035 = ct{13};
t1039 = ct{14};
t104 = ct{15};
t1044 = ct{16};
t1047 = ct{17};
t1049 = ct{18};
t1055 = ct{19};
t1058 = ct{20};
t106 = ct{21};
t1065 = ct{22};
t1066 = ct{23};
t1067 = ct{24};
t107 = ct{25};
t1070 = ct{26};
t1071 = ct{27};
t108 = ct{28};
t1080 = ct{29};
t1083 = ct{30};
t1084 = ct{31};
t1089 = ct{32};
t109 = ct{33};
t1092 = ct{34};
t110 = ct{35};
t1104 = ct{36};
t1105 = ct{37};
t1108 = ct{38};
t111 = ct{39};
t1110 = ct{40};
t1112 = ct{41};
t1113 = ct{42};
t1114 = ct{43};
t1115 = ct{44};
t112 = ct{45};
t1121 = ct{46};
t1123 = ct{47};
t1124 = ct{48};
t1126 = ct{49};
t113 = ct{50};
t1137 = ct{51};
t114 = ct{52};
t1145 = ct{53};
t1148 = ct{54};
t115 = ct{55};
t1150 = ct{56};
t1154 = ct{57};
t1158 = ct{58};
t1159 = ct{59};
t1162 = ct{60};
t1166 = ct{61};
t1167 = ct{62};
t117 = ct{63};
t1170 = ct{64};
t1176 = ct{65};
t1177 = ct{66};
t1178 = ct{67};
t1179 = ct{68};
t118 = ct{69};
t1180 = ct{70};
t1184 = ct{71};
t1185 = ct{72};
t1189 = ct{73};
t1190 = ct{74};
t1192 = ct{75};
t1193 = ct{76};
t1194 = ct{77};
t1196 = ct{78};
t1197 = ct{79};
t1198 = ct{80};
t1199 = ct{81};
t120 = ct{82};
t1202 = ct{83};
t1203 = ct{84};
t1204 = ct{85};
t1205 = ct{86};
t1207 = ct{87};
t1208 = ct{88};
t121 = ct{89};
t1210 = ct{90};
t1212 = ct{91};
t1214 = ct{92};
t1217 = ct{93};
t1218 = ct{94};
t1219 = ct{95};
t122 = ct{96};
t1220 = ct{97};
t1221 = ct{98};
t1222 = ct{99};
t1223 = ct{100};
t1229 = ct{101};
t123 = ct{102};
t1230 = ct{103};
t1232 = ct{104};
t1234 = ct{105};
t1235 = ct{106};
t1236 = ct{107};
t124 = ct{108};
t125 = ct{109};
t126 = ct{110};
t127 = ct{111};
t128 = ct{112};
t1284 = ct{113};
t1285 = ct{114};
t1286 = ct{115};
t1287 = ct{116};
t1288 = ct{117};
t1289 = ct{118};
t129 = ct{119};
t1290 = ct{120};
t1293 = ct{121};
t1299 = ct{122};
t130 = ct{123};
t1300 = ct{124};
t1301 = ct{125};
t1302 = ct{126};
t1303 = ct{127};
t1305 = ct{128};
t1306 = ct{129};
t1307 = ct{130};
t1308 = ct{131};
t1309 = ct{132};
t1311 = ct{133};
t1312 = ct{134};
t1313 = ct{135};
t1315 = ct{136};
t1316 = ct{137};
t1317 = ct{138};
t1318 = ct{139};
t1319 = ct{140};
t132 = ct{141};
t1320 = ct{142};
t1321 = ct{143};
t1322 = ct{144};
t1323 = ct{145};
t1324 = ct{146};
t1328 = ct{147};
t133 = ct{148};
t1333 = ct{149};
t1336 = ct{150};
t1337 = ct{151};
t1338 = ct{152};
t1339 = ct{153};
t134 = ct{154};
t1340 = ct{155};
t1341 = ct{156};
t1342 = ct{157};
t1343 = ct{158};
t1346 = ct{159};
t1347 = ct{160};
t1348 = ct{161};
t1349 = ct{162};
t135 = ct{163};
t1350 = ct{164};
t1351 = ct{165};
t1354 = ct{166};
t1355 = ct{167};
t1356 = ct{168};
t1357 = ct{169};
t1358 = ct{170};
t136 = ct{171};
t1360 = ct{172};
t1361 = ct{173};
t1362 = ct{174};
t1363 = ct{175};
t1366 = ct{176};
t1367 = ct{177};
t1368 = ct{178};
t1369 = ct{179};
t137 = ct{180};
t1378 = ct{181};
t138 = ct{182};
t1384 = ct{183};
t1385 = ct{184};
t1386 = ct{185};
t1387 = ct{186};
t139 = ct{187};
t1392 = ct{188};
t1393 = ct{189};
t1394 = ct{190};
t1395 = ct{191};
t1396 = ct{192};
t1399 = ct{193};
t14 = ct{194};
t1400 = ct{195};
t1425 = ct{196};
t1427 = ct{197};
t1428 = ct{198};
t1429 = ct{199};
t1433 = ct{200};
t1434 = ct{201};
t1435 = ct{202};
t1438 = ct{203};
t144 = ct{204};
t145 = ct{205};
t146 = ct{206};
t147 = ct{207};
t148 = ct{208};
t149 = ct{209};
t15 = ct{210};
t150 = ct{211};
t151 = ct{212};
t152 = ct{213};
t153 = ct{214};
t156 = ct{215};
t157 = ct{216};
t158 = ct{217};
t16 = ct{218};
t160 = ct{219};
t161 = ct{220};
t162 = ct{221};
t163 = ct{222};
t164 = ct{223};
t165 = ct{224};
t166 = ct{225};
t167 = ct{226};
t168 = ct{227};
t169 = ct{228};
t17 = ct{229};
t170 = ct{230};
t171 = ct{231};
t172 = ct{232};
t173 = ct{233};
t174 = ct{234};
t175 = ct{235};
t176 = ct{236};
t177 = ct{237};
t178 = ct{238};
t18 = ct{239};
t180 = ct{240};
t181 = ct{241};
t182 = ct{242};
t185 = ct{243};
t186 = ct{244};
t188 = ct{245};
t189 = ct{246};
t19 = ct{247};
t190 = ct{248};
t191 = ct{249};
t192 = ct{250};
t195 = ct{251};
t196 = ct{252};
t197 = ct{253};
t198 = ct{254};
t2 = ct{255};
t20 = ct{256};
t200 = ct{257};
t201 = ct{258};
t202 = ct{259};
t203 = ct{260};
t204 = ct{261};
t205 = ct{262};
t207 = ct{263};
t208 = ct{264};
t209 = ct{265};
t21 = ct{266};
t210 = ct{267};
t211 = ct{268};
t212 = ct{269};
t216 = ct{270};
t217 = ct{271};
t218 = ct{272};
t219 = ct{273};
t22 = ct{274};
t220 = ct{275};
t221 = ct{276};
t223 = ct{277};
t224 = ct{278};
t225 = ct{279};
t226 = ct{280};
t227 = ct{281};
t229 = ct{282};
t23 = ct{283};
t230 = ct{284};
t231 = ct{285};
t233 = ct{286};
t236 = ct{287};
t237 = ct{288};
t238 = ct{289};
t239 = ct{290};
t24 = ct{291};
t240 = ct{292};
t241 = ct{293};
t242 = ct{294};
t243 = ct{295};
t244 = ct{296};
t245 = ct{297};
t246 = ct{298};
t247 = ct{299};
t25 = ct{300};
t250 = ct{301};
t251 = ct{302};
t252 = ct{303};
t255 = ct{304};
t256 = ct{305};
t257 = ct{306};
t258 = ct{307};
t259 = ct{308};
t26 = ct{309};
t260 = ct{310};
t261 = ct{311};
t262 = ct{312};
t263 = ct{313};
t264 = ct{314};
t265 = ct{315};
t266 = ct{316};
t267 = ct{317};
t269 = ct{318};
t27 = ct{319};
t270 = ct{320};
t271 = ct{321};
t272 = ct{322};
t273 = ct{323};
t274 = ct{324};
t275 = ct{325};
t276 = ct{326};
t277 = ct{327};
t279 = ct{328};
t28 = ct{329};
t280 = ct{330};
t281 = ct{331};
t282 = ct{332};
t283 = ct{333};
t285 = ct{334};
t286 = ct{335};
t289 = ct{336};
t293 = ct{337};
t294 = ct{338};
t295 = ct{339};
t296 = ct{340};
t297 = ct{341};
t298 = ct{342};
t299 = ct{343};
t3 = ct{344};
t30 = ct{345};
t301 = ct{346};
t302 = ct{347};
t303 = ct{348};
t304 = ct{349};
t305 = ct{350};
t306 = ct{351};
t307 = ct{352};
t308 = ct{353};
t309 = ct{354};
t31 = ct{355};
t310 = ct{356};
t311 = ct{357};
t312 = ct{358};
t313 = ct{359};
t314 = ct{360};
t315 = ct{361};
t316 = ct{362};
t318 = ct{363};
t319 = ct{364};
t32 = ct{365};
t320 = ct{366};
t321 = ct{367};
t322 = ct{368};
t323 = ct{369};
t324 = ct{370};
t325 = ct{371};
t326 = ct{372};
t328 = ct{373};
t329 = ct{374};
t33 = ct{375};
t330 = ct{376};
t331 = ct{377};
t332 = ct{378};
t333 = ct{379};
t338 = ct{380};
t339 = ct{381};
t34 = ct{382};
t340 = ct{383};
t341 = ct{384};
t342 = ct{385};
t343 = ct{386};
t344 = ct{387};
t345 = ct{388};
t346 = ct{389};
t348 = ct{390};
t349 = ct{391};
t35 = ct{392};
t350 = ct{393};
t355 = ct{394};
t358 = ct{395};
t359 = ct{396};
t36 = ct{397};
t360 = ct{398};
t363 = ct{399};
t364 = ct{400};
t365 = ct{401};
t366 = ct{402};
t368 = ct{403};
t369 = ct{404};
t370 = ct{405};
t371 = ct{406};
t372 = ct{407};
t373 = ct{408};
t374 = ct{409};
t376 = ct{410};
t377 = ct{411};
t378 = ct{412};
t38 = ct{413};
t381 = ct{414};
t382 = ct{415};
t384 = ct{416};
t385 = ct{417};
t386 = ct{418};
t388 = ct{419};
t389 = ct{420};
t39 = ct{421};
t390 = ct{422};
t391 = ct{423};
t392 = ct{424};
t393 = ct{425};
t396 = ct{426};
t397 = ct{427};
t398 = ct{428};
t4 = ct{429};
t403 = ct{430};
t404 = ct{431};
t405 = ct{432};
t406 = ct{433};
t407 = ct{434};
t408 = ct{435};
t410 = ct{436};
t411 = ct{437};
t412 = ct{438};
t413 = ct{439};
t414 = ct{440};
t415 = ct{441};
t419 = ct{442};
t42 = ct{443};
t420 = ct{444};
t421 = ct{445};
t422 = ct{446};
t423 = ct{447};
t424 = ct{448};
t425 = ct{449};
t426 = ct{450};
t427 = ct{451};
t428 = ct{452};
t43 = ct{453};
t430 = ct{454};
t431 = ct{455};
t432 = ct{456};
t433 = ct{457};
t434 = ct{458};
t435 = ct{459};
t437 = ct{460};
t438 = ct{461};
t439 = ct{462};
t44 = ct{463};
t440 = ct{464};
t441 = ct{465};
t442 = ct{466};
t444 = ct{467};
t445 = ct{468};
t446 = ct{469};
t448 = ct{470};
t449 = ct{471};
t45 = ct{472};
t450 = ct{473};
t451 = ct{474};
t452 = ct{475};
t453 = ct{476};
t454 = ct{477};
t455 = ct{478};
t456 = ct{479};
t457 = ct{480};
t458 = ct{481};
t459 = ct{482};
t46 = ct{483};
t460 = ct{484};
t461 = ct{485};
t462 = ct{486};
t463 = ct{487};
t464 = ct{488};
t465 = ct{489};
t466 = ct{490};
t467 = ct{491};
t468 = ct{492};
t469 = ct{493};
t47 = ct{494};
t470 = ct{495};
t471 = ct{496};
t472 = ct{497};
t473 = ct{498};
t474 = ct{499};
t475 = ct{500};
t476 = ct{501};
t477 = ct{502};
t478 = ct{503};
t479 = ct{504};
t48 = ct{505};
t480 = ct{506};
t481 = ct{507};
t482 = ct{508};
t483 = ct{509};
t484 = ct{510};
t485 = ct{511};
t486 = ct{512};
t487 = ct{513};
t488 = ct{514};
t489 = ct{515};
t490 = ct{516};
t491 = ct{517};
t492 = ct{518};
t493 = ct{519};
t494 = ct{520};
t495 = ct{521};
t496 = ct{522};
t497 = ct{523};
t498 = ct{524};
t499 = ct{525};
t5 = ct{526};
t50 = ct{527};
t500 = ct{528};
t501 = ct{529};
t502 = ct{530};
t503 = ct{531};
t504 = ct{532};
t505 = ct{533};
t506 = ct{534};
t507 = ct{535};
t508 = ct{536};
t509 = ct{537};
t51 = ct{538};
t510 = ct{539};
t511 = ct{540};
t514 = ct{541};
t515 = ct{542};
t516 = ct{543};
t519 = ct{544};
t52 = ct{545};
t520 = ct{546};
t521 = ct{547};
t522 = ct{548};
t528 = ct{549};
t53 = ct{550};
t531 = ct{551};
t532 = ct{552};
t533 = ct{553};
t537 = ct{554};
t54 = ct{555};
t545 = ct{556};
t547 = ct{557};
t548 = ct{558};
t550 = ct{559};
t553 = ct{560};
t554 = ct{561};
t555 = ct{562};
t557 = ct{563};
t559 = ct{564};
t56 = ct{565};
t560 = ct{566};
t561 = ct{567};
t562 = ct{568};
t566 = ct{569};
t568 = ct{570};
t57 = ct{571};
t570 = ct{572};
t58 = ct{573};
t582 = ct{574};
t583 = ct{575};
t584 = ct{576};
t585 = ct{577};
t589 = ct{578};
t59 = ct{579};
t590 = ct{580};
t591 = ct{581};
t592 = ct{582};
t595 = ct{583};
t597 = ct{584};
t599 = ct{585};
t6 = ct{586};
t60 = ct{587};
t600 = ct{588};
t601 = ct{589};
t605 = ct{590};
t606 = ct{591};
t607 = ct{592};
t608 = ct{593};
t609 = ct{594};
t619 = ct{595};
t620 = ct{596};
t621 = ct{597};
t622 = ct{598};
t628 = ct{599};
t63 = ct{600};
t635 = ct{601};
t636 = ct{602};
t638 = ct{603};
t64 = ct{604};
t640 = ct{605};
t641 = ct{606};
t642 = ct{607};
t643 = ct{608};
t645 = ct{609};
t646 = ct{610};
t648 = ct{611};
t649 = ct{612};
t65 = ct{613};
t654 = ct{614};
t655 = ct{615};
t656 = ct{616};
t657 = ct{617};
t659 = ct{618};
t660 = ct{619};
t663 = ct{620};
t664 = ct{621};
t665 = ct{622};
t666 = ct{623};
t667 = ct{624};
t668 = ct{625};
t669 = ct{626};
t67 = ct{627};
t670 = ct{628};
t672 = ct{629};
t673 = ct{630};
t674 = ct{631};
t675 = ct{632};
t676 = ct{633};
t677 = ct{634};
t678 = ct{635};
t679 = ct{636};
t68 = ct{637};
t681 = ct{638};
t682 = ct{639};
t683 = ct{640};
t684 = ct{641};
t685 = ct{642};
t686 = ct{643};
t687 = ct{644};
t689 = ct{645};
t69 = ct{646};
t691 = ct{647};
t692 = ct{648};
t693 = ct{649};
t694 = ct{650};
t7 = ct{651};
t70 = ct{652};
t702 = ct{653};
t704 = ct{654};
t705 = ct{655};
t707 = ct{656};
t708 = ct{657};
t71 = ct{658};
t710 = ct{659};
t711 = ct{660};
t712 = ct{661};
t713 = ct{662};
t714 = ct{663};
t715 = ct{664};
t716 = ct{665};
t717 = ct{666};
t718 = ct{667};
t719 = ct{668};
t72 = ct{669};
t720 = ct{670};
t721 = ct{671};
t722 = ct{672};
t723 = ct{673};
t724 = ct{674};
t725 = ct{675};
t726 = ct{676};
t728 = ct{677};
t73 = ct{678};
t736 = ct{679};
t738 = ct{680};
t740 = ct{681};
t741 = ct{682};
t742 = ct{683};
t743 = ct{684};
t744 = ct{685};
t745 = ct{686};
t746 = ct{687};
t747 = ct{688};
t749 = ct{689};
t75 = ct{690};
t750 = ct{691};
t751 = ct{692};
t755 = ct{693};
t756 = ct{694};
t757 = ct{695};
t758 = ct{696};
t759 = ct{697};
t76 = ct{698};
t762 = ct{699};
t763 = ct{700};
t764 = ct{701};
t766 = ct{702};
t768 = ct{703};
t77 = ct{704};
t770 = ct{705};
t771 = ct{706};
t772 = ct{707};
t773 = ct{708};
t774 = ct{709};
t775 = ct{710};
t776 = ct{711};
t777 = ct{712};
t778 = ct{713};
t78 = ct{714};
t781 = ct{715};
t782 = ct{716};
t783 = ct{717};
t784 = ct{718};
t785 = ct{719};
t786 = ct{720};
t787 = ct{721};
t789 = ct{722};
t79 = ct{723};
t790 = ct{724};
t791 = ct{725};
t792 = ct{726};
t793 = ct{727};
t794 = ct{728};
t796 = ct{729};
t797 = ct{730};
t798 = ct{731};
t799 = ct{732};
t80 = ct{733};
t800 = ct{734};
t801 = ct{735};
t802 = ct{736};
t806 = ct{737};
t807 = ct{738};
t808 = ct{739};
t809 = ct{740};
t81 = ct{741};
t812 = ct{742};
t813 = ct{743};
t816 = ct{744};
t817 = ct{745};
t818 = ct{746};
t819 = ct{747};
t82 = ct{748};
t820 = ct{749};
t821 = ct{750};
t822 = ct{751};
t823 = ct{752};
t824 = ct{753};
t825 = ct{754};
t826 = ct{755};
t827 = ct{756};
t828 = ct{757};
t829 = ct{758};
t830 = ct{759};
t831 = ct{760};
t832 = ct{761};
t833 = ct{762};
t836 = ct{763};
t837 = ct{764};
t838 = ct{765};
t839 = ct{766};
t84 = ct{767};
t840 = ct{768};
t841 = ct{769};
t844 = ct{770};
t845 = ct{771};
t846 = ct{772};
t85 = ct{773};
t850 = ct{774};
t851 = ct{775};
t852 = ct{776};
t853 = ct{777};
t854 = ct{778};
t855 = ct{779};
t857 = ct{780};
t86 = ct{781};
t860 = ct{782};
t861 = ct{783};
t863 = ct{784};
t864 = ct{785};
t866 = ct{786};
t867 = ct{787};
t869 = ct{788};
t874 = ct{789};
t875 = ct{790};
t876 = ct{791};
t877 = ct{792};
t878 = ct{793};
t882 = ct{794};
t883 = ct{795};
t887 = ct{796};
t889 = ct{797};
t89 = ct{798};
t890 = ct{799};
t896 = ct{800};
t897 = ct{801};
t898 = ct{802};
t90 = ct{803};
t900 = ct{804};
t901 = ct{805};
t902 = ct{806};
t903 = ct{807};
t904 = ct{808};
t905 = ct{809};
t906 = ct{810};
t908 = ct{811};
t909 = ct{812};
t91 = ct{813};
t913 = ct{814};
t92 = ct{815};
t920 = ct{816};
t921 = ct{817};
t923 = ct{818};
t924 = ct{819};
t929 = ct{820};
t93 = ct{821};
t938 = ct{822};
t939 = ct{823};
t94 = ct{824};
t946 = ct{825};
t95 = ct{826};
t952 = ct{827};
t954 = ct{828};
t956 = ct{829};
t957 = ct{830};
t96 = ct{831};
t963 = ct{832};
t964 = ct{833};
t97 = ct{834};
t972 = ct{835};
t975 = ct{836};
t977 = ct{837};
t98 = ct{838};
t983 = ct{839};
t986 = ct{840};
t988 = ct{841};
t99 = ct{842};
t996 = ct{843};
t998 = ct{844};
t1237 = -t1219;
t1238 = -t1220;
t1242 = t16.*t17.*t50.*t200.*-4.075691174875038e+36i;
t1243 = t200.*t448;
t1246 = t16.*t22.*t50.*t200.*-4.075691174875038e+36i;
t1247 = t200.*t449;
t1248 = t200.*t450;
t1249 = t200.*t451;
t1252 = t200.*t453;
t1253 = t200.*t454;
t1254 = t16.*t17.*t18.*t50.*t200.*-6.099194893302011e+33i;
t1255 = t21.*t22.*t50.*t200.*1.595073594941899e+37i;
t1256 = t17.*t21.*t23.*t50.*t200.*-6.099194893302011e+33i;
t1265 = t16.*t18.*t50.*t200.*-6.789225223739216e+36i;
t1267 = t18.*t21.*t50.*t200.*-6.789225223739216e+36i;
t1269 = t21.*t200.*7.152220999552773e+52;
t1273 = t200.*t472;
t1274 = t200.*t476;
t1275 = t200.*t477;
t1276 = t200.*t478;
t1277 = t200.*t481;
t1278 = t200.*t482;
t1279 = t200.*t483;
t1280 = t200.*t484;
t1291 = t16.*t17.*t18.*t50.*t200.*-1.249115114148252e+37i;
t1292 = t22.*t200.*3.147052781374869e+48;
t1294 = t16.*t18.*t22.*t50.*t200.*-1.249115114148252e+37i;
t1295 = t16.*t17.*t23.*t50.*t200.*-6.789225223739216e+36i;
t1297 = t16.*t22.*t23.*t50.*t200.*-6.789225223739216e+36i;
t1298 = t18.*t21.*t200.*1.223038087510652e+53;
t1327 = t21.*t23.*t200.*2.250205745048369e+53;
t1329 = t17.*t21.*t200.*1.871019782761396e+48;
t1334 = t17.*t200.*1.253396129822139e+50;
t1335 = -t1284;
t1344 = -t1288;
t1345 = -t1289;
t1352 = -t1293;
t1370 = -t1302;
t1371 = -t1303;
t1373 = t16.*t200.*7.917244648613035e+49;
t1374 = -t1306;
t1375 = -t1308;
t1376 = -t1309;
t1379 = -t1312;
t1380 = -t1313;
t1389 = -t1315;
t1397 = -t1318;
t1398 = -t1321;
t1404 = -t1333;
t1405 = -t1336;
t1406 = -t1339;
t1407 = -t1340;
t1408 = -t1341;
t1409 = -t1346;
t1410 = -t1347;
t1411 = -t1350;
t1412 = -t1351;
t1413 = t16.*t22.*t23.*t200.*1.223038087510652e+53;
t1414 = -t1355;
t1415 = -t1356;
t1416 = -t1357;
t1417 = -t1358;
t1419 = -t1361;
t1420 = -t1362;
t1421 = -t1363;
t1424 = -t1369;
t1430 = t16.*t18.*t22.*t200.*2.250205745048369e+53;
t1436 = -t1384;
t1440 = -t1396;
t1441 = -t1400;
t1443 = t22.*t23.*t200.*1.004467008511696e+50;
t1445 = t21.*t22.*t200.*7.451825938264896e+49;
t1446 = t18.*t22.*t200.*1.848067902664462e+50;
t1447 = -t1435;
t1448 = -t1438;
t1454 = t16.*t50.*t189.*5.673626844500105e-17;
t1455 = t21.*t50.*t189.*5.673626844500105e-17;
t1456 = t17.*t50.*t189.*9.543032792050485e-17;
t1458 = t22.*t50.*t189.*9.543032792050485e-17;
t1470 = t17.*t21.*t23.*t200.*5.971865661673106e+49;
t1473 = t17.*t18.*t21.*t200.*1.098733273949399e+50;
t1474 = t26.*t50.*t202.*5.673626844500105e-17;
t1475 = t32.*t50.*t202.*5.673626844500105e-17;
t1477 = t27.*t50.*t202.*9.543032792050485e-17;
t1478 = t33.*t50.*t202.*9.543032792050485e-17;
t1480 = t16.*t50.*t189.*6.489053738789607e-19;
t1481 = t21.*t50.*t189.*6.489053738789607e-19;
t1483 = t16.*t50.*t189.*1.092459456231154e-21;
t1488 = t17.*t50.*t189.*5.725819675230291e-19;
t1490 = t16.*t50.*t189.*7.194245199571015e-21;
t1491 = t50.*t200.*6.804240878490729e+18i;
t1492 = t22.*t50.*t189.*5.725819675230291e-19;
t1493 = t21.*t50.*t189.*7.194245199571015e-21;
t1496 = t16.*t17.*t50.*t189.*1.384627967837559e-18;
t1497 = t16.*t22.*t50.*t189.*1.384627967837559e-18;
t1498 = t17.*t21.*t50.*t189.*1.384627967837559e-18;
t1500 = t16.*t22.*t50.*t189.*6.313682909819818e-19;
t1501 = t21.*t22.*t50.*t189.*6.313682909819818e-19;
t1503 = t32.*t50.*t202.*6.489053738789607e-19;
t1509 = t16.*t17.*t50.*t189.*6.313682909819818e-19;
t1511 = t21.*t50.*t189.*6.88338275267597e-23;
t1513 = t27.*t50.*t202.*5.725819675230291e-19;
t1514 = t33.*t50.*t202.*5.725819675230291e-19;
t1515 = t32.*t50.*t202.*7.194245199571015e-21;
t1517 = t16.*t50.*t189.*6.417111286793897e-19;
t1518 = t21.*t50.*t189.*3.597122599785507e-22;
t1519 = t16.*t50.*t189.*7.183142969324763e-22;
t1520 = t21.*t50.*t189.*8.693046282814975e-22;
t1521 = t21.*t50.*t189.*7.183142969324763e-22;
t1523 = t16.*t23.*t50.*t200.*1.354293320444013e+18i;
t1524 = t16.*t18.*t50.*t200.*7.360892737071442e+17i;
t1528 = t17.*t18.*t50.*t200.*2.277919560321538e+18i;
t1530 = t17.*t23.*t50.*t200.*1.238101177498716e+18i;
t1537 = t26.*t50.*t202.*7.183142969324763e-22;
t1538 = t16.*t50.*t189.*5.673626844500105e-25;
t1539 = t21.*t50.*t189.*5.673626844500105e-25;
t1541 = t18.*t21.*t22.*t50.*t200.*1.354293320444013e+18i;
t1542 = t21.*t22.*t23.*t50.*t200.*7.360892737071442e+17i;
t1545 = t17.*t50.*t189.*9.543032792050485e-25;
t1546 = t22.*t50.*t189.*9.543032792050485e-25;
t1560 = t14.*t15.*t188.*1.374006108587572e-3;
t1561 = t14.*t20.*t188.*1.374006108587572e-3;
t1562 = t15.*t19.*t188.*1.374006108587572e-3;
t1563 = t19.*t20.*t188.*1.374006108587572e-3;
t1566 = t19.*t20.*t188.*6.463878411896211e-3;
t1567 = t14.*t15.*t188.*2.311076443710702e-3;
t1570 = t14.*t20.*t188.*2.311076443710702e-3;
t1571 = t15.*t19.*t188.*2.311076443710702e-3;
t1573 = t19.*t20.*t188.*2.311076443710702e-3;
t1576 = t14.*t15.*t188.*6.463878411896211e-3;
t1577 = t14.*t20.*t188.*6.463878411896211e-3;
t1578 = t15.*t19.*t188.*6.463878411896211e-3;
t1581 = t14.*t15.*t188.*1.087223487536e-2;
t1582 = t201.*8.618586366948822e-4;
t1584 = t14.*t20.*t188.*1.087223487536e-2;
t1585 = t15.*t19.*t188.*1.087223487536e-2;
t1586 = t19.*t20.*t188.*1.087223487536e-2;
t1587 = t14.*t15.*t188.*2.550195842399381e-2;
t1589 = t14.*t20.*t188.*2.550195842399381e-2;
t1590 = t15.*t19.*t188.*2.550195842399381e-2;
t1591 = t19.*t20.*t188.*2.550195842399381e-2;
t1593 = t201.*5.135409293037228e-4;
t1607 = t14.*t15.*t188.*4.289426008649035e-2;
t1608 = t14.*t20.*t188.*4.289426008649035e-2;
t1609 = t15.*t19.*t188.*4.289426008649035e-2;
t1611 = t19.*t20.*t188.*4.289426008649035e-2;
t1614 = t24.*t25.*t201.*6.463878411896211e-3;
t1615 = t24.*t31.*t201.*6.463878411896211e-3;
t1616 = t25.*t30.*t201.*6.463878411896211e-3;
t1617 = t30.*t31.*t201.*6.463878411896211e-3;
t1621 = t27.*t201.*5.316843277159623e-5;
t1623 = t33.*t201.*5.316843277159623e-5;
t1624 = t27.*t201.*1.166015146360021e-4;
t1625 = t33.*t201.*1.166015146360021e-4;
t1638 = t24.*t25.*t201.*1.087223487536e-2;
t1648 = t24.*t31.*t201.*1.087223487536e-2;
t1649 = t25.*t30.*t201.*1.087223487536e-2;
t1660 = t30.*t31.*t201.*1.087223487536e-2;
t1686 = t24.*t25.*t201.*2.550195842399381e-2;
t1688 = t24.*t31.*t201.*2.550195842399381e-2;
t1689 = t25.*t30.*t201.*2.550195842399381e-2;
t1690 = t30.*t31.*t201.*2.550195842399381e-2;
t1695 = t16.*t50.*t200.*1.553819674864718e+37i;
t1700 = t24.*t31.*t201.*4.289426008649035e-2;
t1701 = t25.*t30.*t201.*4.289426008649035e-2;
t1702 = t30.*t31.*t201.*4.289426008649035e-2;
t1750 = t24.*t25.*t201.*4.289426008649035e-2;
t1765 = t16.*t23.*t50.*t200.*4.888570919953966e+37i;
t1780 = t16.*t18.*t50.*t200.*2.657049668350291e+37i;
t1782 = t21.*t50.*t200.*1.720021026545681e+34i;
t1795 = t18.*t21.*t22.*t50.*t200.*4.888570919953966e+37i;
t1796 = t16.*t17.*t50.*t200.*4.064789595703988e+32i;
t1797 = t21.*t22.*t23.*t50.*t200.*2.657049668350291e+37i;
t1798 = t16.*t22.*t50.*t200.*1.618908833671003e+34i;
t1807 = t16.*t17.*t18.*t50.*t200.*2.386997519508773e+34i;
t1817 = t16.*t17.*t23.*t50.*t200.*1.297387533374166e+34i;
t1863 = t16.*t50.*t189.*(t42-t43).*(-1.232595164407831e-32);
t1865 = t21.*t50.*t189.*(t42-t43).*(-1.232595164407831e-32);
t1868 = (t16.*t50.*t189.*(t42-t43))./8.112963841460668e+31;
t1870 = t50.*t189.*1.930470600839964e-18;
t1871 = t16.*t50.*t189.*5.582848814988104e-22;
t1872 = t21.*t50.*t189.*5.582848814988104e-22;
t1873 = t50.*t189.*3.311325901843639e-18;
t1874 = t50.*t189.*5.241796502683603e-18;
t1875 = t50.*t189.*5.241796502683603e-18;
t1876 = t50.*t202.*1.930470600839964e-18;
t1877 = t50.*t202.*3.311325901843639e-18;
t1879 = t50.*t202.*5.241796502683603e-18;
t1880 = t35.*t50.*t189.*2.899421184450801e-17;
t1881 = t36.*t50.*t189.*2.899421184450801e-17;
t1882 = t17.*t50.*t189.*5.426989146380022e-19;
t1883 = t17.*t50.*t189.*5.426989146380022e-19;
t1884 = t22.*t50.*t189.*5.426989146380022e-19;
t1886 = t16.*t50.*t189.*3.31613276532711e-19;
t1887 = t21.*t50.*t189.*3.31613276532711e-19;
t1889 = t17.*t50.*t189.*1.190170786299927e-18;
t1890 = t22.*t50.*t189.*1.190170786299927e-18;
t1891 = t22.*t50.*t189.*1.190170786299927e-18;
t1894 = t16.*t50.*t189.*3.676510195236068e-21;
t1895 = t16.*t50.*t189.*3.676510195236068e-21;
t1897 = t21.*t50.*t189.*3.676510195236068e-21;
t1898 = t16.*t50.*t189.*4.442449819243582e-22;
t1899 = t21.*t50.*t189.*4.442449819243582e-22;
t1901 = t35.*t50.*t189.*8.202809061800765e-17;
t1902 = t36.*t50.*t189.*8.202809061800765e-17;
t1903 = t16.*t50.*t189.*3.517648643590065e-23;
t1904 = t21.*t50.*t189.*3.517648643590065e-23;
t1907 = t50.*t189.*3.091942624624357e-22;
t1909 = t16.*t17.*t50.*t189.*7.075931802640439e-19;
t1914 = t16.*t22.*t50.*t189.*7.075931802640439e-19;
t1915 = t17.*t21.*t50.*t189.*7.075931802640439e-19;
t1916 = t17.*t21.*t50.*t189.*7.075931802640439e-19;
t1917 = t16.*t50.*t189.*1.838255097618034e-22;
t1919 = t21.*t50.*t189.*1.838255097618034e-22;
t1920 = t16.*t17.*t50.*t189.*3.226512155691387e-19;
t1922 = t16.*t22.*t50.*t189.*3.226512155691387e-19;
t1923 = t27.*t50.*t202.*5.426989146380022e-19;
t1924 = t21.*t22.*t50.*t189.*3.226512155691387e-19;
t1925 = t21.*t22.*t50.*t189.*3.226512155691387e-19;
t1926 = t33.*t50.*t202.*5.426989146380022e-19;
t1927 = t26.*t50.*t202.*3.31613276532711e-19;
t1928 = t50.*t189.*2.967883198327701e-22;
t1929 = t32.*t50.*t202.*3.31613276532711e-19;
t1930 = t27.*t50.*t202.*1.190170786299927e-18;
t1931 = t33.*t50.*t202.*1.190170786299927e-18;
t1936 = t16.*t50.*t189.*3.279367663374749e-19;
t1937 = t21.*t50.*t189.*3.279367663374749e-19;
t1940 = t16.*t50.*t189.*3.670836568391568e-22;
t1941 = t38.*t50.*t202.*2.899421184450801e-17;
t1942 = t21.*t50.*t189.*3.670836568391568e-22;
t1943 = t39.*t50.*t202.*2.899421184450801e-17;
t1947 = t17.*t50.*t189.*2.988305288502687e-20;
t1948 = t22.*t50.*t189.*2.988305288502687e-20;
t1949 = t26.*t50.*t202.*3.676510195236068e-21;
t1950 = t32.*t50.*t202.*3.676510195236068e-21;
t1951 = t17.*t50.*t189.*5.439528691468777e-23;
t1952 = t22.*t50.*t189.*5.439528691468777e-23;
t1953 = t17.*t50.*t189.*9.733893447891495e-23;
t1956 = t22.*t50.*t189.*9.733893447891495e-23;
t1958 = t38.*t50.*t202.*8.202809061800765e-17;
t1959 = t39.*t50.*t202.*8.202809061800765e-17;
t1960 = t26.*t50.*t202.*1.875105520197095e-20;
t1961 = t32.*t50.*t202.*1.875105520197095e-20;
t1965 = t17.*t50.*t189.*2.290327870092116e-23;
t1966 = t22.*t50.*t189.*2.290327870092116e-23;
t1967 = t26.*t50.*t202.*3.670836568391568e-22;
t1968 = t32.*t50.*t202.*3.670836568391568e-22;
t1970 = t27.*t50.*t202.*2.988305288502687e-20;
t1971 = t33.*t50.*t202.*2.988305288502687e-20;
t1975 = t14.*t17.*t20.*t21.*t50.*t189.*3.226512155691387e-19;
t1977 = t15.*t17.*t19.*t21.*t50.*t189.*3.226512155691387e-19;
t1982 = t17.*t19.*t20.*t21.*t50.*t189.*3.226512155691387e-19;
t1991 = t26.*t50.*t202.*7.825108561121397e-23;
t1997 = t32.*t50.*t202.*7.825108561121397e-23;
t2017 = t14.*t15.*t21.*t22.*t50.*t189.*7.075931802640439e-19;
t2021 = t14.*t20.*t21.*t22.*t50.*t189.*7.075931802640439e-19;
t2022 = t15.*t19.*t21.*t22.*t50.*t189.*7.075931802640439e-19;
t2024 = t17.*t50.*t189.*3.817213116820194e-24;
t2025 = t19.*t20.*t21.*t22.*t50.*t189.*7.075931802640439e-19;
t2027 = t14.*t15.*t17.*t21.*t50.*t189.*3.226512155691387e-19;
t2028 = t22.*t50.*t189.*3.817213116820194e-24;
t2029 = t14.*t15.*t21.*t22.*t50.*t189.*(-3.226512155691387e-19);
t2030 = t14.*t16.*t20.*t22.*t50.*t189.*(-3.226512155691387e-19);
t2032 = t15.*t16.*t19.*t22.*t50.*t189.*(-3.226512155691387e-19);
t2034 = t26.*t50.*t202.*2.075672598245148e-23;
t2035 = t26.*t33.*t50.*t202.*6.867329764181918e-21;
t2038 = t32.*t50.*t202.*2.075672598245148e-23;
t2039 = t32.*t33.*t50.*t202.*6.867329764181918e-21;
t2043 = t14.*t15.*t21.*t22.*t50.*t189.*(-5.426989146380022e-19);
t2044 = t14.*t16.*t20.*t22.*t50.*t189.*(-5.426989146380022e-19);
t2045 = t15.*t16.*t19.*t22.*t50.*t189.*(-5.426989146380022e-19);
t2049 = t14.*t20.*t21.*t22.*t50.*t189.*(-5.426989146380022e-19);
t2050 = t15.*t19.*t21.*t22.*t50.*t189.*(-5.426989146380022e-19);
t2051 = t16.*t19.*t20.*t22.*t50.*t189.*(-5.426989146380022e-19);
t2052 = t17.*t19.*t20.*t21.*t50.*t189.*(-5.426989146380022e-19);
t2054 = t14.*t15.*t16.*t17.*t50.*t189.*(-1.190170786299927e-18);
t2055 = t26.*t27.*t50.*t202.*1.506045994337235e-20;
t2056 = t26.*t33.*t50.*t202.*1.506045994337235e-20;
t2057 = t27.*t32.*t50.*t202.*1.506045994337235e-20;
t2058 = t17.*t19.*t20.*t21.*t50.*t189.*(-1.190170786299927e-18);
t2059 = t19.*t20.*t21.*t22.*t50.*t189.*(-1.190170786299927e-18);
t2061 = t14.*t17.*t20.*t21.*t50.*t189.*(-7.075931802640439e-19);
t2062 = t15.*t17.*t19.*t21.*t50.*t189.*(-7.075931802640439e-19);
t2063 = t16.*t17.*t19.*t20.*t50.*t189.*(-7.075931802640439e-19);
t2069 = t17.*t19.*t20.*t21.*t50.*t189.*(-7.075931802640439e-19);
t2075 = t14.*t15.*t16.*t22.*t50.*t189.*(-3.226512155691387e-19);
t2077 = t26.*t27.*t50.*t202.*6.867329764181918e-21;
t2080 = t14.*t15.*t16.*t50.*t189.*6.174342216456664e-22;
t2081 = t14.*t20.*t21.*t50.*t189.*(-3.670836568391568e-22);
t2082 = t15.*t19.*t21.*t50.*t189.*(-3.670836568391568e-22);
t2083 = t16.*t19.*t20.*t50.*t189.*(-3.670836568391568e-22);
t2084 = t14.*t15.*t21.*t50.*t189.*6.174342216456664e-22;
t2085 = t14.*t16.*t20.*t50.*t189.*6.174342216456664e-22;
t2086 = t15.*t16.*t19.*t50.*t189.*6.174342216456664e-22;
t2087 = t19.*t20.*t21.*t50.*t189.*(-3.670836568391568e-22);
t2088 = t32.*t50.*t202.*7.813032776304851e-24;
t2089 = t14.*t20.*t21.*t50.*t189.*6.174342216456664e-22;
t2090 = t15.*t19.*t21.*t50.*t189.*6.174342216456664e-22;
t2091 = t16.*t19.*t20.*t50.*t189.*6.174342216456664e-22;
t2092 = t19.*t20.*t21.*t50.*t189.*6.174342216456664e-22;
t2093 = t26.*t50.*t202.*6.979827775532854e-21;
t2096 = t14.*t15.*t16.*t50.*t189.*5.515892039870764e-19;
t2097 = t14.*t15.*t21.*t50.*t189.*5.515892039870764e-19;
t2098 = t14.*t16.*t20.*t50.*t189.*5.515892039870764e-19;
t2099 = t15.*t16.*t19.*t50.*t189.*5.515892039870764e-19;
t2100 = t14.*t20.*t21.*t50.*t189.*5.515892039870764e-19;
t2101 = t15.*t19.*t21.*t50.*t189.*5.515892039870764e-19;
t2102 = t16.*t19.*t20.*t50.*t189.*5.515892039870764e-19;
t2103 = t19.*t20.*t21.*t50.*t189.*5.515892039870764e-19;
t2104 = t14.*t15.*t16.*t50.*t189.*(-3.279367663374749e-19);
t2105 = t19.*t20.*t21.*t50.*t189.*(-3.279367663374749e-19);
t2117 = t24.*t25.*t201.*7.713980286110892e-6;
t2118 = t24.*t31.*t201.*7.713980286110892e-6;
t2119 = t25.*t30.*t201.*7.713980286110892e-6;
t2120 = t30.*t31.*t201.*7.713980286110892e-6;
t2121 = t24.*t25.*t201.*4.586198809426854e-6;
t2122 = t24.*t31.*t201.*4.586198809426854e-6;
t2123 = t25.*t30.*t201.*4.586198809426854e-6;
t2124 = t30.*t31.*t201.*4.586198809426854e-6;
t2131 = t30.*t31.*t201.*1.867830746966542e-4;
t2138 = t24.*t25.*t201.*1.867830746966542e-4;
t2139 = t24.*t31.*t201.*1.867830746966542e-4;
t2140 = t25.*t30.*t201.*1.867830746966542e-4;
t2147 = t24.*t25.*t201.*4.665565775347468e-4;
t2149 = t24.*t31.*t201.*4.665565775347468e-4;
t2150 = t25.*t30.*t201.*4.665565775347468e-4;
t2151 = t24.*t25.*t201.*2.773822515819383e-4;
t2152 = t30.*t31.*t201.*4.665565775347468e-4;
t2153 = t24.*t25.*t201.*3.141688827417478e-4;
t2154 = t24.*t31.*t201.*2.773822515819383e-4;
t2155 = t25.*t30.*t201.*2.773822515819383e-4;
t2156 = t24.*t31.*t201.*3.141688827417478e-4;
t2157 = t25.*t30.*t201.*3.141688827417478e-4;
t2158 = t30.*t31.*t201.*2.773822515819383e-4;
t2159 = t30.*t31.*t201.*3.141688827417478e-4;
t2294 = t16.*t50.*t189.*(t42-t43).*(-7.204296868834178e-35);
t2296 = t21.*t50.*t189.*(t42-t43).*(-7.204296868834178e-35);
t2299 = t16.*t50.*t189.*(t42-t43).*(-7.987216665362745e-37);
t2300 = t16.*t50.*t189.*(t42-t43).*7.204296868834178e-35;
t2302 = t21.*t50.*t189.*(t42-t43).*(-7.987216665362745e-37);
t2303 = t21.*t50.*t189.*(t42-t43).*7.204296868834178e-35;
t2305 = t35.*t50.*t189.*2.492226411042213e-17;
t2306 = t36.*t50.*t189.*2.492226411042213e-17;
t2308 = t35.*t50.*t189.*3.691525655515653e-19;
t2309 = t36.*t50.*t189.*3.691525655515653e-19;
t2310 = t16.*t50.*t189.*(t42-t43).*7.987216665362745e-37;
t2313 = t21.*t50.*t189.*(t42-t43).*(-7.974890713718666e-38);
t2314 = t14.*t15.*t50.*t189.*1.525453217729535e-19;
t2315 = t14.*t20.*t50.*t189.*1.525453217729535e-19;
t2316 = t15.*t19.*t50.*t189.*1.525453217729535e-19;
t2317 = t35.*t50.*t189.*4.191921502353519e-17;
t2318 = t19.*t20.*t50.*t189.*1.525453217729535e-19;
t2319 = t36.*t50.*t189.*4.191921502353519e-17;
t2322 = t35.*t50.*t189.*3.487329940320384e-18;
t2323 = t36.*t50.*t189.*3.487329940320384e-18;
t2324 = t16.*t50.*t189.*(t42-t43).*(-7.974890713718666e-38);
t2325 = t21.*t50.*t189.*(t42-t43).*7.974890713718666e-38;
t2326 = t14.*t15.*t50.*t189.*7.176346641264665e-19;
t2327 = t14.*t20.*t50.*t189.*7.176346641264665e-19;
t2328 = t15.*t19.*t50.*t189.*7.176346641264665e-19;
t2329 = t19.*t20.*t50.*t189.*7.176346641264665e-19;
t2330 = t14.*t15.*t50.*t189.*2.565810279476446e-19;
t2331 = t14.*t20.*t50.*t189.*2.565810279476446e-19;
t2332 = t15.*t19.*t50.*t189.*2.565810279476446e-19;
t2334 = t19.*t20.*t50.*t189.*2.565810279476446e-19;
t2339 = t16.*t50.*t189.*(t42-t43).*7.974890713718666e-38;
t2340 = t50.*t202.*5.701449638003928e-20;
t2345 = t38.*t50.*t202.*2.492226411042213e-17;
t2346 = t39.*t50.*t202.*2.492226411042213e-17;
t2348 = t14.*t15.*t50.*t189.*1.207060548775729e-18;
t2349 = t35.*t50.*t189.*1.89580370025077e-18;
t2352 = t14.*t20.*t50.*t189.*1.207060548775729e-18;
t2353 = t15.*t19.*t50.*t189.*1.207060548775729e-18;
t2354 = t36.*t50.*t189.*1.89580370025077e-18;
t2357 = t19.*t20.*t50.*t189.*1.207060548775729e-18;
t2358 = t38.*t50.*t202.*3.691525655515653e-19;
t2359 = t14.*t15.*t50.*t189.*2.83128614153514e-18;
t2360 = t39.*t50.*t202.*3.691525655515653e-19;
t2361 = t14.*t20.*t50.*t189.*2.83128614153514e-18;
t2362 = t15.*t19.*t50.*t189.*2.83128614153514e-18;
t2364 = t19.*t20.*t50.*t189.*2.83128614153514e-18;
t2365 = t14.*t20.*t50.*t189.*4.762219517228144e-18;
t2366 = t15.*t19.*t50.*t189.*4.762219517228144e-18;
t2367 = t19.*t20.*t50.*t189.*4.762219517228144e-18;
t2374 = t35.*t50.*t189.*5.383133640571155e-18;
t2378 = t36.*t50.*t189.*5.383133640571155e-18;
t2382 = t38.*t50.*t202.*4.191921502353519e-17;
t2383 = t39.*t50.*t202.*4.191921502353519e-17;
t2391 = t38.*t50.*t202.*3.487329940320384e-18;
t2392 = t39.*t50.*t202.*3.487329940320384e-18;
t2393 = t14.*t15.*t50.*t189.*4.762219517228144e-18;
t2402 = t24.*t25.*t50.*t202.*7.176346641264665e-19;
t2404 = t24.*t31.*t50.*t202.*7.176346641264665e-19;
t2405 = t25.*t30.*t50.*t202.*7.176346641264665e-19;
t2406 = t30.*t31.*t50.*t202.*7.176346641264665e-19;
t2407 = t26.*t50.*t202.*3.998903374256319e-23;
t2409 = t27.*t50.*t202.*5.902881824626087e-21;
t2411 = t33.*t50.*t202.*1.294536862550567e-20;
t2415 = t30.*t31.*t50.*t202.*2.83128614153514e-18;
t2416 = t14.*t15.*t21.*t50.*t189.*1.675871243454932e-19;
t2417 = t14.*t20.*t21.*t50.*t189.*1.675871243454932e-19;
t2418 = t15.*t19.*t21.*t50.*t189.*1.675871243454932e-19;
t2420 = t19.*t20.*t21.*t50.*t189.*1.675871243454932e-19;
t2426 = t14.*t15.*t16.*t22.*t50.*t189.*2.773380719257578e-19;
t2427 = t14.*t15.*t16.*t17.*t50.*t189.*3.616047923242029e-19;
t2428 = t24.*t25.*t50.*t202.*1.207060548775729e-18;
t2429 = t14.*t16.*t20.*t22.*t50.*t189.*2.773380719257578e-19;
t2430 = t15.*t16.*t19.*t22.*t50.*t189.*2.773380719257578e-19;
t2431 = t14.*t16.*t17.*t20.*t50.*t189.*3.616047923242029e-19;
t2432 = t15.*t16.*t17.*t19.*t50.*t189.*3.616047923242029e-19;
t2433 = t24.*t31.*t50.*t202.*1.207060548775729e-18;
t2434 = t25.*t30.*t50.*t202.*1.207060548775729e-18;
t2435 = t14.*t15.*t16.*t17.*t50.*t189.*6.082187788323819e-19;
t2436 = t16.*t19.*t20.*t22.*t50.*t189.*2.773380719257578e-19;
t2437 = t16.*t17.*t19.*t20.*t50.*t189.*3.616047923242029e-19;
t2438 = t30.*t31.*t50.*t202.*1.207060548775729e-18;
t2439 = t14.*t15.*t16.*t22.*t50.*t189.*1.648860235700588e-19;
t2440 = t14.*t16.*t17.*t20.*t50.*t189.*6.082187788323819e-19;
t2441 = t15.*t16.*t17.*t19.*t50.*t189.*6.082187788323819e-19;
t2442 = t14.*t16.*t20.*t22.*t50.*t189.*1.648860235700588e-19;
t2443 = t15.*t16.*t19.*t22.*t50.*t189.*1.648860235700588e-19;
t2444 = t16.*t17.*t19.*t20.*t50.*t189.*6.082187788323819e-19;
t2446 = t16.*t19.*t20.*t22.*t50.*t189.*1.648860235700588e-19;
t2447 = t24.*t25.*t50.*t202.*2.83128614153514e-18;
t2448 = t24.*t31.*t50.*t202.*2.83128614153514e-18;
t2449 = t25.*t30.*t50.*t202.*2.83128614153514e-18;
t2451 = t26.*t27.*t50.*t202.*7.696420262413979e-21;
t2452 = t26.*t33.*t50.*t202.*7.696420262413979e-21;
t2453 = t27.*t32.*t50.*t202.*7.696420262413979e-21;
t2454 = t27.*t32.*t50.*t202.*7.69642026241398e-21;
t2455 = t26.*t50.*t202.*3.566935413776081e-21;
t2456 = t24.*t25.*t50.*t202.*4.762219517228144e-18;
t2457 = t32.*t50.*t202.*3.566935413776081e-21;
t2459 = t24.*t31.*t50.*t202.*4.762219517228144e-18;
t2460 = t25.*t30.*t50.*t202.*4.762219517228144e-18;
t2461 = t30.*t31.*t50.*t202.*4.762219517228144e-18;
t2463 = t14.*t15.*t16.*t50.*t189.*1.875925506339668e-22;
t2466 = t14.*t16.*t20.*t50.*t189.*1.875925506339668e-22;
t2467 = t15.*t16.*t19.*t50.*t189.*1.875925506339668e-22;
t2469 = t16.*t19.*t20.*t50.*t189.*1.875925506339668e-22;
t2471 = t38.*t50.*t202.*5.383133640571155e-18;
t2475 = t39.*t50.*t202.*5.383133640571155e-18;
t2482 = t26.*t27.*t50.*t202.*3.509445006623964e-21;
t2483 = t26.*t33.*t50.*t202.*3.509445006623964e-21;
t2484 = t32.*t33.*t50.*t202.*3.509445006623964e-21;
t2485 = t32.*t33.*t50.*t202.*3.509445006623964e-21;
t2486 = t14.*t15.*t21.*t50.*t189.*2.818813198306831e-19;
t2487 = t14.*t20.*t21.*t50.*t189.*2.818813198306831e-19;
t2488 = t15.*t19.*t21.*t50.*t189.*2.818813198306831e-19;
t2491 = t19.*t20.*t21.*t50.*t189.*2.818813198306831e-19;
t2495 = t14.*t15.*t16.*t50.*t189.*3.155304201896394e-22;
t2498 = t14.*t16.*t20.*t50.*t189.*3.155304201896394e-22;
t2499 = t15.*t16.*t19.*t50.*t189.*3.155304201896394e-22;
t2505 = t16.*t19.*t20.*t50.*t189.*3.155304201896394e-22;
t2512 = t26.*t50.*t202.*3.992732227073824e-24;
t2513 = t32.*t50.*t202.*3.992732227073824e-24;
t2515 = t189.*t202.*2.393852475650798e-6;
t2529 = t189.*t202.*2.297802839282093e-6;
t2541 = t24.*t25.*t27.*t32.*t50.*t202.*3.509445006623964e-21;
t2544 = t24.*t27.*t31.*t32.*t50.*t202.*3.509445006623964e-21;
t2546 = t25.*t27.*t30.*t32.*t50.*t202.*3.509445006623964e-21;
t2551 = t27.*t30.*t31.*t32.*t50.*t202.*3.509445006623964e-21;
t2560 = t24.*t25.*t32.*t33.*t50.*t202.*7.696420262413979e-21;
t2567 = t24.*t31.*t32.*t33.*t50.*t202.*7.696420262413979e-21;
t2568 = t25.*t30.*t32.*t33.*t50.*t202.*7.696420262413979e-21;
t2573 = t30.*t31.*t32.*t33.*t50.*t202.*7.696420262413979e-21;
t2577 = t24.*t25.*t26.*t33.*t50.*t202.*(-3.509445006623964e-21);
t2579 = t24.*t26.*t31.*t33.*t50.*t202.*(-3.509445006623964e-21);
t2581 = t25.*t26.*t30.*t33.*t50.*t202.*(-3.509445006623964e-21);
t2586 = t24.*t25.*t26.*t33.*t50.*t202.*5.902881824626087e-21;
t2587 = t24.*t25.*t27.*t32.*t50.*t202.*5.902881824626087e-21;
t2588 = t24.*t25.*t26.*t27.*t50.*t202.*1.294536862550567e-20;
t2593 = t24.*t25.*t32.*t33.*t50.*t202.*5.902881824626087e-21;
t2594 = t24.*t26.*t31.*t33.*t50.*t202.*5.902881824626087e-21;
t2595 = t24.*t27.*t31.*t32.*t50.*t202.*5.902881824626087e-21;
t2596 = t25.*t26.*t30.*t33.*t50.*t202.*5.902881824626087e-21;
t2597 = t25.*t27.*t30.*t32.*t50.*t202.*5.902881824626087e-21;
t2599 = t24.*t25.*t27.*t32.*t50.*t202.*1.294536862550567e-20;
t2600 = t24.*t26.*t27.*t31.*t50.*t202.*1.294536862550567e-20;
t2601 = t25.*t26.*t27.*t30.*t50.*t202.*1.294536862550567e-20;
t2603 = t30.*t31.*t32.*t33.*t50.*t202.*(-3.509445006623964e-21);
t2605 = t24.*t31.*t32.*t33.*t50.*t202.*5.902881824626087e-21;
t2606 = t25.*t30.*t32.*t33.*t50.*t202.*5.902881824626087e-21;
t2607 = t26.*t30.*t31.*t33.*t50.*t202.*5.902881824626087e-21;
t2608 = t27.*t30.*t31.*t32.*t50.*t202.*5.902881824626087e-21;
t2609 = t24.*t25.*t26.*t50.*t202.*5.999580612847032e-21;
t2610 = t24.*t25.*t27.*t32.*t50.*t202.*(-7.696420262413979e-21);
t2611 = t24.*t25.*t32.*t33.*t50.*t202.*1.294536862550567e-20;
t2612 = t24.*t27.*t31.*t32.*t50.*t202.*1.294536862550567e-20;
t2613 = t25.*t27.*t30.*t32.*t50.*t202.*1.294536862550567e-20;
t2614 = t26.*t27.*t30.*t31.*t50.*t202.*1.294536862550567e-20;
t2616 = t30.*t31.*t32.*t33.*t50.*t202.*5.902881824626087e-21;
t2617 = t24.*t25.*t32.*t50.*t202.*5.999580612847032e-21;
t2618 = t24.*t26.*t31.*t50.*t202.*5.999580612847032e-21;
t2619 = t25.*t26.*t30.*t50.*t202.*5.999580612847032e-21;
t2620 = t24.*t27.*t31.*t32.*t50.*t202.*(-7.696420262413979e-21);
t2621 = t25.*t27.*t30.*t32.*t50.*t202.*(-7.696420262413979e-21);
t2622 = t26.*t27.*t30.*t31.*t50.*t202.*(-7.696420262413979e-21);
t2623 = t24.*t31.*t32.*t33.*t50.*t202.*1.294536862550567e-20;
t2624 = t25.*t30.*t32.*t33.*t50.*t202.*1.294536862550567e-20;
tau_c = ft_3({t100,t1000,t1001,t1002,t1003,t1006,t1008,t101,t1019,t102,t103,t1030,t1035,t1039,t104,t1044,t1047,t1049,t1055,t1058,t106,t1065,t1066,t1067,t107,t1070,t1071,t108,t1080,t1083,t1084,t1089,t109,t1092,t110,t1104,t1105,t1108,t111,t1110,t1112,t1113,t1114,t1115,t112,t1121,t1123,t1124,t1126,t113,t1137,t114,t1145,t1148,t115,t1150,t1154,t1158,t1159,t1162,t1166,t1167,t117,t1170,t1176,t1177,t1178,t1179,t118,t1180,t1184,t1185,t1189,t1190,t1192,t1193,t1194,t1196,t1197,t1198,t1199,t120,t1202,t1203,t1204,t1205,t1207,t1208,t121,t1210,t1212,t1214,t1217,t1218,t1219,t122,t1220,t1221,t1222,t1223,t1229,t123,t1230,t1232,t1234,t1235,t1236,t1237,t1238,t124,t1242,t1246,t1247,t1248,t125,t1252,t1253,t1254,t1255,t1256,t126,t1265,t1267,t1269,t127,t1277,t1278,t128,t1280,t1285,t1286,t1287,t1288,t1289,t129,t1290,t1291,t1292,t1294,t1295,t1297,t1298,t1299,t130,t1300,t1301,t1302,t1303,t1305,t1307,t1311,t1316,t1317,t1319,t132,t1320,t1322,t1323,t1324,t1327,t1328,t1329,t133,t1334,t1335,t1336,t1337,t1338,t134,t1342,t1343,t1344,t1345,t1348,t1349,t135,t1350,t1351,t1352,t1354,t136,t1360,t1366,t1367,t1368,t1369,t137,t1370,t1371,t1373,t1374,t1375,t1376,t1378,t1379,t138,t1380,t1385,t1386,t1387,t1389,t139,t1392,t1393,t1394,t1395,t1396,t1397,t1398,t1399,t14,t1404,t1405,t1406,t1407,t1408,t1409,t1410,t1411,t1412,t1413,t1414,t1415,t1416,t1417,t1419,t1420,t1421,t1424,t1425,t1427,t1428,t1429,t1430,t1433,t1434,t1435,t1436,t144,t1440,t1441,t1443,t1445,t1446,t1447,t1448,t145,t1454,t1455,t1456,t1458,t146,t147,t1470,t1473,t1474,t1475,t1477,t1478,t148,t1480,t1481,t1483,t1488,t149,t1490,t1491,t1492,t1493,t1496,t1497,t1498,t15,t150,t1500,t1501,t1503,t1509,t151,t1511,t1513,t1514,t1515,t1517,t1518,t1519,t152,t1520,t1521,t1523,t1524,t1528,t153,t1530,t1537,t1538,t1539,t1541,t1542,t1545,t1546,t156,t1560,t1561,t1562,t1563,t1566,t1567,t157,t1570,t1571,t1573,t1576,t1577,t1578,t158,t1581,t1582,t1584,t1585,t1586,t1587,t1589,t1590,t1591,t1593,t16,t160,t1607,t1608,t1609,t161,t1611,t1614,t1615,t1616,t1617,t162,t1621,t1623,t1624,t1625,t163,t1638,t164,t1648,t1649,t165,t166,t1660,t167,t168,t1686,t1688,t1689,t169,t1690,t1695,t17,t170,t1700,t1701,t1702,t171,t172,t173,t174,t175,t1750,t176,t1765,t177,t178,t1780,t1782,t1795,t1796,t1797,t1798,t18,t180,t1807,t181,t1817,t182,t185,t186,t1865,t1868,t1870,t1871,t1872,t1873,t1874,t1875,t1876,t1877,t1879,t188,t1880,t1881,t1882,t1883,t1884,t1886,t1887,t1889,t189,t1890,t1891,t1894,t1895,t1897,t1898,t1899,t19,t190,t1901,t1902,t1903,t1904,t1907,t1909,t191,t1914,t1915,t1916,t1917,t1919,t192,t1920,t1922,t1923,t1924,t1925,t1926,t1927,t1928,t1929,t1930,t1931,t1936,t1937,t1940,t1941,t1942,t1943,t1947,t1948,t1949,t195,t1950,t1951,t1952,t1953,t1956,t1958,t1959,t196,t1960,t1961,t1965,t1966,t1967,t1968,t197,t1970,t1971,t1975,t1977,t198,t1982,t1991,t1997,t2,t20,t201,t2017,t202,t2021,t2022,t2024,t2025,t2027,t2028,t2029,t203,t2030,t2032,t2034,t2035,t2038,t2039,t204,t2043,t2044,t2045,t2049,t205,t2050,t2051,t2052,t2054,t2055,t2056,t2057,t2058,t2059,t2061,t2062,t2063,t2069,t207,t2075,t2077,t208,t2080,t2081,t2082,t2083,t2084,t2085,t2086,t2087,t2088,t2089,t209,t2090,t2091,t2092,t2093,t2096,t2097,t2098,t2099,t21,t210,t2100,t2101,t2102,t2103,t2104,t2105,t211,t2117,t2118,t2119,t212,t2120,t2121,t2122,t2123,t2124,t2131,t2138,t2139,t2140,t2147,t2149,t2150,t2151,t2152,t2153,t2154,t2155,t2156,t2157,t2158,t2159,t216,t217,t218,t219,t22,t220,t221,t223,t224,t225,t226,t227,t229,t2294,t2296,t2299,t23,t230,t2300,t2302,t2303,t2305,t2306,t2308,t2309,t231,t2310,t2313,t2314,t2315,t2316,t2317,t2318,t2319,t2322,t2323,t2324,t2325,t2326,t2327,t2328,t2329,t233,t2330,t2331,t2332,t2334,t2339,t2340,t2345,t2346,t2348,t2349,t2352,t2353,t2354,t2357,t2358,t2359,t236,t2360,t2361,t2362,t2364,t2365,t2366,t2367,t237,t2374,t2378,t238,t2382,t2383,t239,t2391,t2392,t2393,t24,t240,t2402,t2404,t2405,t2406,t2407,t2409,t241,t2411,t2415,t2416,t2417,t2418,t242,t2420,t2426,t2427,t2428,t2429,t243,t2430,t2431,t2432,t2433,t2434,t2435,t2436,t2437,t2438,t2439,t244,t2440,t2441,t2442,t2443,t2444,t2446,t2447,t2448,t2449,t245,t2451,t2452,t2453,t2454,t2455,t2456,t2457,t2459,t246,t2460,t2461,t2463,t2466,t2467,t2469,t247,t2471,t2475,t2482,t2483,t2484,t2485,t2486,t2487,t2488,t2491,t2495,t2498,t2499,t25,t250,t2505,t251,t2512,t2513,t2515,t252,t2529,t2541,t2544,t2546,t255,t2551,t256,t2560,t2567,t2568,t257,t2573,t2577,t2579,t258,t2581,t2586,t2587,t2588,t259,t2593,t2594,t2595,t2596,t2597,t2599,t26,t260,t2600,t2601,t2603,t2605,t2606,t2607,t2608,t2609,t261,t2610,t2611,t2612,t2613,t2614,t2616,t2617,t2618,t2619,t262,t2620,t2621,t2622,t2623,t2624,t263,t264,t265,t266,t267,t269,t27,t270,t271,t272,t273,t274,t275,t276,t277,t279,t28,t280,t281,t282,t283,t285,t286,t289,t293,t294,t295,t296,t297,t298,t299,t3,t30,t301,t302,t303,t304,t305,t306,t307,t308,t309,t31,t310,t311,t312,t313,t314,t315,t316,t318,t319,t32,t320,t321,t322,t323,t324,t325,t326,t328,t329,t33,t330,t331,t332,t333,t338,t339,t34,t340,t341,t342,t343,t344,t345,t346,t348,t349,t35,t350,t355,t358,t359,t36,t360,t363,t364,t365,t366,t368,t369,t370,t371,t372,t373,t374,t376,t377,t378,t38,t381,t382,t384,t385,t386,t388,t389,t39,t390,t391,t392,t393,t396,t397,t398,t4,t403,t404,t405,t406,t407,t408,t410,t411,t412,t413,t414,t415,t419,t42,t420,t421,t422,t423,t424,t425,t426,t427,t428,t43,t430,t431,t432,t433,t434,t435,t437,t438,t439,t44,t440,t441,t442,t444,t445,t446,t448,t45,t451,t452,t455,t456,t457,t458,t459,t46,t460,t461,t462,t463,t464,t465,t466,t467,t468,t469,t47,t470,t471,t472,t473,t474,t475,t476,t477,t478,t479,t48,t480,t483,t485,t486,t487,t488,t489,t490,t491,t492,t493,t494,t495,t496,t497,t498,t499,t5,t50,t500,t501,t502,t503,t504,t505,t506,t507,t508,t509,t51,t510,t511,t514,t515,t516,t519,t52,t520,t521,t522,t528,t53,t531,t532,t533,t537,t54,t545,t547,t548,t550,t553,t554,t555,t557,t559,t56,t560,t561,t562,t566,t568,t57,t570,t58,t582,t583,t584,t585,t589,t59,t590,t591,t592,t595,t597,t599,t6,t60,t600,t601,t605,t606,t607,t608,t609,t619,t620,t621,t622,t628,t63,t635,t636,t638,t64,t640,t641,t642,t643,t645,t646,t648,t649,t65,t654,t655,t656,t657,t659,t660,t663,t664,t665,t666,t667,t668,t669,t67,t670,t672,t673,t674,t675,t676,t677,t678,t679,t68,t681,t682,t683,t684,t685,t686,t687,t689,t69,t691,t692,t693,t694,t7,t70,t702,t704,t705,t707,t708,t71,t710,t711,t712,t713,t714,t715,t716,t717,t718,t719,t72,t720,t721,t722,t723,t724,t725,t726,t728,t73,t736,t738,t740,t741,t742,t743,t744,t745,t746,t747,t749,t75,t750,t751,t755,t756,t757,t758,t759,t76,t762,t763,t764,t766,t768,t77,t770,t771,t772,t773,t774,t775,t776,t777,t778,t78,t781,t782,t783,t784,t785,t786,t787,t789,t79,t790,t791,t792,t793,t794,t796,t797,t798,t799,t80,t800,t801,t802,t806,t807,t808,t809,t81,t812,t813,t816,t817,t818,t819,t82,t820,t821,t822,t823,t824,t825,t826,t827,t828,t829,t830,t831,t832,t833,t836,t837,t838,t839,t84,t840,t841,t844,t845,t846,t85,t850,t851,t852,t853,t854,t855,t857,t86,t860,t861,t863,t864,t866,t867,t869,t874,t875,t876,t877,t878,t882,t883,t887,t889,t89,t890,t896,t897,t898,t90,t900,t901,t902,t903,t904,t905,t906,t908,t909,t91,t913,t92,t920,t921,t923,t924,t929,t93,t938,t939,t94,t946,t95,t952,t954,t956,t957,t96,t963,t964,t97,t972,t975,t977,t98,t983,t986,t988,t99,t996,t998});
end
function tau_c = ft_3(ct)
t100 = ct{1};
t1000 = ct{2};
t1001 = ct{3};
t1002 = ct{4};
t1003 = ct{5};
t1006 = ct{6};
t1008 = ct{7};
t101 = ct{8};
t1019 = ct{9};
t102 = ct{10};
t103 = ct{11};
t1030 = ct{12};
t1035 = ct{13};
t1039 = ct{14};
t104 = ct{15};
t1044 = ct{16};
t1047 = ct{17};
t1049 = ct{18};
t1055 = ct{19};
t1058 = ct{20};
t106 = ct{21};
t1065 = ct{22};
t1066 = ct{23};
t1067 = ct{24};
t107 = ct{25};
t1070 = ct{26};
t1071 = ct{27};
t108 = ct{28};
t1080 = ct{29};
t1083 = ct{30};
t1084 = ct{31};
t1089 = ct{32};
t109 = ct{33};
t1092 = ct{34};
t110 = ct{35};
t1104 = ct{36};
t1105 = ct{37};
t1108 = ct{38};
t111 = ct{39};
t1110 = ct{40};
t1112 = ct{41};
t1113 = ct{42};
t1114 = ct{43};
t1115 = ct{44};
t112 = ct{45};
t1121 = ct{46};
t1123 = ct{47};
t1124 = ct{48};
t1126 = ct{49};
t113 = ct{50};
t1137 = ct{51};
t114 = ct{52};
t1145 = ct{53};
t1148 = ct{54};
t115 = ct{55};
t1150 = ct{56};
t1154 = ct{57};
t1158 = ct{58};
t1159 = ct{59};
t1162 = ct{60};
t1166 = ct{61};
t1167 = ct{62};
t117 = ct{63};
t1170 = ct{64};
t1176 = ct{65};
t1177 = ct{66};
t1178 = ct{67};
t1179 = ct{68};
t118 = ct{69};
t1180 = ct{70};
t1184 = ct{71};
t1185 = ct{72};
t1189 = ct{73};
t1190 = ct{74};
t1192 = ct{75};
t1193 = ct{76};
t1194 = ct{77};
t1196 = ct{78};
t1197 = ct{79};
t1198 = ct{80};
t1199 = ct{81};
t120 = ct{82};
t1202 = ct{83};
t1203 = ct{84};
t1204 = ct{85};
t1205 = ct{86};
t1207 = ct{87};
t1208 = ct{88};
t121 = ct{89};
t1210 = ct{90};
t1212 = ct{91};
t1214 = ct{92};
t1217 = ct{93};
t1218 = ct{94};
t1219 = ct{95};
t122 = ct{96};
t1220 = ct{97};
t1221 = ct{98};
t1222 = ct{99};
t1223 = ct{100};
t1229 = ct{101};
t123 = ct{102};
t1230 = ct{103};
t1232 = ct{104};
t1234 = ct{105};
t1235 = ct{106};
t1236 = ct{107};
t1237 = ct{108};
t1238 = ct{109};
t124 = ct{110};
t1242 = ct{111};
t1246 = ct{112};
t1247 = ct{113};
t1248 = ct{114};
t125 = ct{115};
t1252 = ct{116};
t1253 = ct{117};
t1254 = ct{118};
t1255 = ct{119};
t1256 = ct{120};
t126 = ct{121};
t1265 = ct{122};
t1267 = ct{123};
t1269 = ct{124};
t127 = ct{125};
t1277 = ct{126};
t1278 = ct{127};
t128 = ct{128};
t1280 = ct{129};
t1285 = ct{130};
t1286 = ct{131};
t1287 = ct{132};
t1288 = ct{133};
t1289 = ct{134};
t129 = ct{135};
t1290 = ct{136};
t1291 = ct{137};
t1292 = ct{138};
t1294 = ct{139};
t1295 = ct{140};
t1297 = ct{141};
t1298 = ct{142};
t1299 = ct{143};
t130 = ct{144};
t1300 = ct{145};
t1301 = ct{146};
t1302 = ct{147};
t1303 = ct{148};
t1305 = ct{149};
t1307 = ct{150};
t1311 = ct{151};
t1316 = ct{152};
t1317 = ct{153};
t1319 = ct{154};
t132 = ct{155};
t1320 = ct{156};
t1322 = ct{157};
t1323 = ct{158};
t1324 = ct{159};
t1327 = ct{160};
t1328 = ct{161};
t1329 = ct{162};
t133 = ct{163};
t1334 = ct{164};
t1335 = ct{165};
t1336 = ct{166};
t1337 = ct{167};
t1338 = ct{168};
t134 = ct{169};
t1342 = ct{170};
t1343 = ct{171};
t1344 = ct{172};
t1345 = ct{173};
t1348 = ct{174};
t1349 = ct{175};
t135 = ct{176};
t1350 = ct{177};
t1351 = ct{178};
t1352 = ct{179};
t1354 = ct{180};
t136 = ct{181};
t1360 = ct{182};
t1366 = ct{183};
t1367 = ct{184};
t1368 = ct{185};
t1369 = ct{186};
t137 = ct{187};
t1370 = ct{188};
t1371 = ct{189};
t1373 = ct{190};
t1374 = ct{191};
t1375 = ct{192};
t1376 = ct{193};
t1378 = ct{194};
t1379 = ct{195};
t138 = ct{196};
t1380 = ct{197};
t1385 = ct{198};
t1386 = ct{199};
t1387 = ct{200};
t1389 = ct{201};
t139 = ct{202};
t1392 = ct{203};
t1393 = ct{204};
t1394 = ct{205};
t1395 = ct{206};
t1396 = ct{207};
t1397 = ct{208};
t1398 = ct{209};
t1399 = ct{210};
t14 = ct{211};
t1404 = ct{212};
t1405 = ct{213};
t1406 = ct{214};
t1407 = ct{215};
t1408 = ct{216};
t1409 = ct{217};
t1410 = ct{218};
t1411 = ct{219};
t1412 = ct{220};
t1413 = ct{221};
t1414 = ct{222};
t1415 = ct{223};
t1416 = ct{224};
t1417 = ct{225};
t1419 = ct{226};
t1420 = ct{227};
t1421 = ct{228};
t1424 = ct{229};
t1425 = ct{230};
t1427 = ct{231};
t1428 = ct{232};
t1429 = ct{233};
t1430 = ct{234};
t1433 = ct{235};
t1434 = ct{236};
t1435 = ct{237};
t1436 = ct{238};
t144 = ct{239};
t1440 = ct{240};
t1441 = ct{241};
t1443 = ct{242};
t1445 = ct{243};
t1446 = ct{244};
t1447 = ct{245};
t1448 = ct{246};
t145 = ct{247};
t1454 = ct{248};
t1455 = ct{249};
t1456 = ct{250};
t1458 = ct{251};
t146 = ct{252};
t147 = ct{253};
t1470 = ct{254};
t1473 = ct{255};
t1474 = ct{256};
t1475 = ct{257};
t1477 = ct{258};
t1478 = ct{259};
t148 = ct{260};
t1480 = ct{261};
t1481 = ct{262};
t1483 = ct{263};
t1488 = ct{264};
t149 = ct{265};
t1490 = ct{266};
t1491 = ct{267};
t1492 = ct{268};
t1493 = ct{269};
t1496 = ct{270};
t1497 = ct{271};
t1498 = ct{272};
t15 = ct{273};
t150 = ct{274};
t1500 = ct{275};
t1501 = ct{276};
t1503 = ct{277};
t1509 = ct{278};
t151 = ct{279};
t1511 = ct{280};
t1513 = ct{281};
t1514 = ct{282};
t1515 = ct{283};
t1517 = ct{284};
t1518 = ct{285};
t1519 = ct{286};
t152 = ct{287};
t1520 = ct{288};
t1521 = ct{289};
t1523 = ct{290};
t1524 = ct{291};
t1528 = ct{292};
t153 = ct{293};
t1530 = ct{294};
t1537 = ct{295};
t1538 = ct{296};
t1539 = ct{297};
t1541 = ct{298};
t1542 = ct{299};
t1545 = ct{300};
t1546 = ct{301};
t156 = ct{302};
t1560 = ct{303};
t1561 = ct{304};
t1562 = ct{305};
t1563 = ct{306};
t1566 = ct{307};
t1567 = ct{308};
t157 = ct{309};
t1570 = ct{310};
t1571 = ct{311};
t1573 = ct{312};
t1576 = ct{313};
t1577 = ct{314};
t1578 = ct{315};
t158 = ct{316};
t1581 = ct{317};
t1582 = ct{318};
t1584 = ct{319};
t1585 = ct{320};
t1586 = ct{321};
t1587 = ct{322};
t1589 = ct{323};
t1590 = ct{324};
t1591 = ct{325};
t1593 = ct{326};
t16 = ct{327};
t160 = ct{328};
t1607 = ct{329};
t1608 = ct{330};
t1609 = ct{331};
t161 = ct{332};
t1611 = ct{333};
t1614 = ct{334};
t1615 = ct{335};
t1616 = ct{336};
t1617 = ct{337};
t162 = ct{338};
t1621 = ct{339};
t1623 = ct{340};
t1624 = ct{341};
t1625 = ct{342};
t163 = ct{343};
t1638 = ct{344};
t164 = ct{345};
t1648 = ct{346};
t1649 = ct{347};
t165 = ct{348};
t166 = ct{349};
t1660 = ct{350};
t167 = ct{351};
t168 = ct{352};
t1686 = ct{353};
t1688 = ct{354};
t1689 = ct{355};
t169 = ct{356};
t1690 = ct{357};
t1695 = ct{358};
t17 = ct{359};
t170 = ct{360};
t1700 = ct{361};
t1701 = ct{362};
t1702 = ct{363};
t171 = ct{364};
t172 = ct{365};
t173 = ct{366};
t174 = ct{367};
t175 = ct{368};
t1750 = ct{369};
t176 = ct{370};
t1765 = ct{371};
t177 = ct{372};
t178 = ct{373};
t1780 = ct{374};
t1782 = ct{375};
t1795 = ct{376};
t1796 = ct{377};
t1797 = ct{378};
t1798 = ct{379};
t18 = ct{380};
t180 = ct{381};
t1807 = ct{382};
t181 = ct{383};
t1817 = ct{384};
t182 = ct{385};
t185 = ct{386};
t186 = ct{387};
t1865 = ct{388};
t1868 = ct{389};
t1870 = ct{390};
t1871 = ct{391};
t1872 = ct{392};
t1873 = ct{393};
t1874 = ct{394};
t1875 = ct{395};
t1876 = ct{396};
t1877 = ct{397};
t1879 = ct{398};
t188 = ct{399};
t1880 = ct{400};
t1881 = ct{401};
t1882 = ct{402};
t1883 = ct{403};
t1884 = ct{404};
t1886 = ct{405};
t1887 = ct{406};
t1889 = ct{407};
t189 = ct{408};
t1890 = ct{409};
t1891 = ct{410};
t1894 = ct{411};
t1895 = ct{412};
t1897 = ct{413};
t1898 = ct{414};
t1899 = ct{415};
t19 = ct{416};
t190 = ct{417};
t1901 = ct{418};
t1902 = ct{419};
t1903 = ct{420};
t1904 = ct{421};
t1907 = ct{422};
t1909 = ct{423};
t191 = ct{424};
t1914 = ct{425};
t1915 = ct{426};
t1916 = ct{427};
t1917 = ct{428};
t1919 = ct{429};
t192 = ct{430};
t1920 = ct{431};
t1922 = ct{432};
t1923 = ct{433};
t1924 = ct{434};
t1925 = ct{435};
t1926 = ct{436};
t1927 = ct{437};
t1928 = ct{438};
t1929 = ct{439};
t1930 = ct{440};
t1931 = ct{441};
t1936 = ct{442};
t1937 = ct{443};
t1940 = ct{444};
t1941 = ct{445};
t1942 = ct{446};
t1943 = ct{447};
t1947 = ct{448};
t1948 = ct{449};
t1949 = ct{450};
t195 = ct{451};
t1950 = ct{452};
t1951 = ct{453};
t1952 = ct{454};
t1953 = ct{455};
t1956 = ct{456};
t1958 = ct{457};
t1959 = ct{458};
t196 = ct{459};
t1960 = ct{460};
t1961 = ct{461};
t1965 = ct{462};
t1966 = ct{463};
t1967 = ct{464};
t1968 = ct{465};
t197 = ct{466};
t1970 = ct{467};
t1971 = ct{468};
t1975 = ct{469};
t1977 = ct{470};
t198 = ct{471};
t1982 = ct{472};
t1991 = ct{473};
t1997 = ct{474};
t2 = ct{475};
t20 = ct{476};
t201 = ct{477};
t2017 = ct{478};
t202 = ct{479};
t2021 = ct{480};
t2022 = ct{481};
t2024 = ct{482};
t2025 = ct{483};
t2027 = ct{484};
t2028 = ct{485};
t2029 = ct{486};
t203 = ct{487};
t2030 = ct{488};
t2032 = ct{489};
t2034 = ct{490};
t2035 = ct{491};
t2038 = ct{492};
t2039 = ct{493};
t204 = ct{494};
t2043 = ct{495};
t2044 = ct{496};
t2045 = ct{497};
t2049 = ct{498};
t205 = ct{499};
t2050 = ct{500};
t2051 = ct{501};
t2052 = ct{502};
t2054 = ct{503};
t2055 = ct{504};
t2056 = ct{505};
t2057 = ct{506};
t2058 = ct{507};
t2059 = ct{508};
t2061 = ct{509};
t2062 = ct{510};
t2063 = ct{511};
t2069 = ct{512};
t207 = ct{513};
t2075 = ct{514};
t2077 = ct{515};
t208 = ct{516};
t2080 = ct{517};
t2081 = ct{518};
t2082 = ct{519};
t2083 = ct{520};
t2084 = ct{521};
t2085 = ct{522};
t2086 = ct{523};
t2087 = ct{524};
t2088 = ct{525};
t2089 = ct{526};
t209 = ct{527};
t2090 = ct{528};
t2091 = ct{529};
t2092 = ct{530};
t2093 = ct{531};
t2096 = ct{532};
t2097 = ct{533};
t2098 = ct{534};
t2099 = ct{535};
t21 = ct{536};
t210 = ct{537};
t2100 = ct{538};
t2101 = ct{539};
t2102 = ct{540};
t2103 = ct{541};
t2104 = ct{542};
t2105 = ct{543};
t211 = ct{544};
t2117 = ct{545};
t2118 = ct{546};
t2119 = ct{547};
t212 = ct{548};
t2120 = ct{549};
t2121 = ct{550};
t2122 = ct{551};
t2123 = ct{552};
t2124 = ct{553};
t2131 = ct{554};
t2138 = ct{555};
t2139 = ct{556};
t2140 = ct{557};
t2147 = ct{558};
t2149 = ct{559};
t2150 = ct{560};
t2151 = ct{561};
t2152 = ct{562};
t2153 = ct{563};
t2154 = ct{564};
t2155 = ct{565};
t2156 = ct{566};
t2157 = ct{567};
t2158 = ct{568};
t2159 = ct{569};
t216 = ct{570};
t217 = ct{571};
t218 = ct{572};
t219 = ct{573};
t22 = ct{574};
t220 = ct{575};
t221 = ct{576};
t223 = ct{577};
t224 = ct{578};
t225 = ct{579};
t226 = ct{580};
t227 = ct{581};
t229 = ct{582};
t2294 = ct{583};
t2296 = ct{584};
t2299 = ct{585};
t23 = ct{586};
t230 = ct{587};
t2300 = ct{588};
t2302 = ct{589};
t2303 = ct{590};
t2305 = ct{591};
t2306 = ct{592};
t2308 = ct{593};
t2309 = ct{594};
t231 = ct{595};
t2310 = ct{596};
t2313 = ct{597};
t2314 = ct{598};
t2315 = ct{599};
t2316 = ct{600};
t2317 = ct{601};
t2318 = ct{602};
t2319 = ct{603};
t2322 = ct{604};
t2323 = ct{605};
t2324 = ct{606};
t2325 = ct{607};
t2326 = ct{608};
t2327 = ct{609};
t2328 = ct{610};
t2329 = ct{611};
t233 = ct{612};
t2330 = ct{613};
t2331 = ct{614};
t2332 = ct{615};
t2334 = ct{616};
t2339 = ct{617};
t2340 = ct{618};
t2345 = ct{619};
t2346 = ct{620};
t2348 = ct{621};
t2349 = ct{622};
t2352 = ct{623};
t2353 = ct{624};
t2354 = ct{625};
t2357 = ct{626};
t2358 = ct{627};
t2359 = ct{628};
t236 = ct{629};
t2360 = ct{630};
t2361 = ct{631};
t2362 = ct{632};
t2364 = ct{633};
t2365 = ct{634};
t2366 = ct{635};
t2367 = ct{636};
t237 = ct{637};
t2374 = ct{638};
t2378 = ct{639};
t238 = ct{640};
t2382 = ct{641};
t2383 = ct{642};
t239 = ct{643};
t2391 = ct{644};
t2392 = ct{645};
t2393 = ct{646};
t24 = ct{647};
t240 = ct{648};
t2402 = ct{649};
t2404 = ct{650};
t2405 = ct{651};
t2406 = ct{652};
t2407 = ct{653};
t2409 = ct{654};
t241 = ct{655};
t2411 = ct{656};
t2415 = ct{657};
t2416 = ct{658};
t2417 = ct{659};
t2418 = ct{660};
t242 = ct{661};
t2420 = ct{662};
t2426 = ct{663};
t2427 = ct{664};
t2428 = ct{665};
t2429 = ct{666};
t243 = ct{667};
t2430 = ct{668};
t2431 = ct{669};
t2432 = ct{670};
t2433 = ct{671};
t2434 = ct{672};
t2435 = ct{673};
t2436 = ct{674};
t2437 = ct{675};
t2438 = ct{676};
t2439 = ct{677};
t244 = ct{678};
t2440 = ct{679};
t2441 = ct{680};
t2442 = ct{681};
t2443 = ct{682};
t2444 = ct{683};
t2446 = ct{684};
t2447 = ct{685};
t2448 = ct{686};
t2449 = ct{687};
t245 = ct{688};
t2451 = ct{689};
t2452 = ct{690};
t2453 = ct{691};
t2454 = ct{692};
t2455 = ct{693};
t2456 = ct{694};
t2457 = ct{695};
t2459 = ct{696};
t246 = ct{697};
t2460 = ct{698};
t2461 = ct{699};
t2463 = ct{700};
t2466 = ct{701};
t2467 = ct{702};
t2469 = ct{703};
t247 = ct{704};
t2471 = ct{705};
t2475 = ct{706};
t2482 = ct{707};
t2483 = ct{708};
t2484 = ct{709};
t2485 = ct{710};
t2486 = ct{711};
t2487 = ct{712};
t2488 = ct{713};
t2491 = ct{714};
t2495 = ct{715};
t2498 = ct{716};
t2499 = ct{717};
t25 = ct{718};
t250 = ct{719};
t2505 = ct{720};
t251 = ct{721};
t2512 = ct{722};
t2513 = ct{723};
t2515 = ct{724};
t252 = ct{725};
t2529 = ct{726};
t2541 = ct{727};
t2544 = ct{728};
t2546 = ct{729};
t255 = ct{730};
t2551 = ct{731};
t256 = ct{732};
t2560 = ct{733};
t2567 = ct{734};
t2568 = ct{735};
t257 = ct{736};
t2573 = ct{737};
t2577 = ct{738};
t2579 = ct{739};
t258 = ct{740};
t2581 = ct{741};
t2586 = ct{742};
t2587 = ct{743};
t2588 = ct{744};
t259 = ct{745};
t2593 = ct{746};
t2594 = ct{747};
t2595 = ct{748};
t2596 = ct{749};
t2597 = ct{750};
t2599 = ct{751};
t26 = ct{752};
t260 = ct{753};
t2600 = ct{754};
t2601 = ct{755};
t2603 = ct{756};
t2605 = ct{757};
t2606 = ct{758};
t2607 = ct{759};
t2608 = ct{760};
t2609 = ct{761};
t261 = ct{762};
t2610 = ct{763};
t2611 = ct{764};
t2612 = ct{765};
t2613 = ct{766};
t2614 = ct{767};
t2616 = ct{768};
t2617 = ct{769};
t2618 = ct{770};
t2619 = ct{771};
t262 = ct{772};
t2620 = ct{773};
t2621 = ct{774};
t2622 = ct{775};
t2623 = ct{776};
t2624 = ct{777};
t263 = ct{778};
t264 = ct{779};
t265 = ct{780};
t266 = ct{781};
t267 = ct{782};
t269 = ct{783};
t27 = ct{784};
t270 = ct{785};
t271 = ct{786};
t272 = ct{787};
t273 = ct{788};
t274 = ct{789};
t275 = ct{790};
t276 = ct{791};
t277 = ct{792};
t279 = ct{793};
t28 = ct{794};
t280 = ct{795};
t281 = ct{796};
t282 = ct{797};
t283 = ct{798};
t285 = ct{799};
t286 = ct{800};
t289 = ct{801};
t293 = ct{802};
t294 = ct{803};
t295 = ct{804};
t296 = ct{805};
t297 = ct{806};
t298 = ct{807};
t299 = ct{808};
t3 = ct{809};
t30 = ct{810};
t301 = ct{811};
t302 = ct{812};
t303 = ct{813};
t304 = ct{814};
t305 = ct{815};
t306 = ct{816};
t307 = ct{817};
t308 = ct{818};
t309 = ct{819};
t31 = ct{820};
t310 = ct{821};
t311 = ct{822};
t312 = ct{823};
t313 = ct{824};
t314 = ct{825};
t315 = ct{826};
t316 = ct{827};
t318 = ct{828};
t319 = ct{829};
t32 = ct{830};
t320 = ct{831};
t321 = ct{832};
t322 = ct{833};
t323 = ct{834};
t324 = ct{835};
t325 = ct{836};
t326 = ct{837};
t328 = ct{838};
t329 = ct{839};
t33 = ct{840};
t330 = ct{841};
t331 = ct{842};
t332 = ct{843};
t333 = ct{844};
t338 = ct{845};
t339 = ct{846};
t34 = ct{847};
t340 = ct{848};
t341 = ct{849};
t342 = ct{850};
t343 = ct{851};
t344 = ct{852};
t345 = ct{853};
t346 = ct{854};
t348 = ct{855};
t349 = ct{856};
t35 = ct{857};
t350 = ct{858};
t355 = ct{859};
t358 = ct{860};
t359 = ct{861};
t36 = ct{862};
t360 = ct{863};
t363 = ct{864};
t364 = ct{865};
t365 = ct{866};
t366 = ct{867};
t368 = ct{868};
t369 = ct{869};
t370 = ct{870};
t371 = ct{871};
t372 = ct{872};
t373 = ct{873};
t374 = ct{874};
t376 = ct{875};
t377 = ct{876};
t378 = ct{877};
t38 = ct{878};
t381 = ct{879};
t382 = ct{880};
t384 = ct{881};
t385 = ct{882};
t386 = ct{883};
t388 = ct{884};
t389 = ct{885};
t39 = ct{886};
t390 = ct{887};
t391 = ct{888};
t392 = ct{889};
t393 = ct{890};
t396 = ct{891};
t397 = ct{892};
t398 = ct{893};
t4 = ct{894};
t403 = ct{895};
t404 = ct{896};
t405 = ct{897};
t406 = ct{898};
t407 = ct{899};
t408 = ct{900};
t410 = ct{901};
t411 = ct{902};
t412 = ct{903};
t413 = ct{904};
t414 = ct{905};
t415 = ct{906};
t419 = ct{907};
t42 = ct{908};
t420 = ct{909};
t421 = ct{910};
t422 = ct{911};
t423 = ct{912};
t424 = ct{913};
t425 = ct{914};
t426 = ct{915};
t427 = ct{916};
t428 = ct{917};
t43 = ct{918};
t430 = ct{919};
t431 = ct{920};
t432 = ct{921};
t433 = ct{922};
t434 = ct{923};
t435 = ct{924};
t437 = ct{925};
t438 = ct{926};
t439 = ct{927};
t44 = ct{928};
t440 = ct{929};
t441 = ct{930};
t442 = ct{931};
t444 = ct{932};
t445 = ct{933};
t446 = ct{934};
t448 = ct{935};
t45 = ct{936};
t451 = ct{937};
t452 = ct{938};
t455 = ct{939};
t456 = ct{940};
t457 = ct{941};
t458 = ct{942};
t459 = ct{943};
t46 = ct{944};
t460 = ct{945};
t461 = ct{946};
t462 = ct{947};
t463 = ct{948};
t464 = ct{949};
t465 = ct{950};
t466 = ct{951};
t467 = ct{952};
t468 = ct{953};
t469 = ct{954};
t47 = ct{955};
t470 = ct{956};
t471 = ct{957};
t472 = ct{958};
t473 = ct{959};
t474 = ct{960};
t475 = ct{961};
t476 = ct{962};
t477 = ct{963};
t478 = ct{964};
t479 = ct{965};
t48 = ct{966};
t480 = ct{967};
t483 = ct{968};
t485 = ct{969};
t486 = ct{970};
t487 = ct{971};
t488 = ct{972};
t489 = ct{973};
t490 = ct{974};
t491 = ct{975};
t492 = ct{976};
t493 = ct{977};
t494 = ct{978};
t495 = ct{979};
t496 = ct{980};
t497 = ct{981};
t498 = ct{982};
t499 = ct{983};
t5 = ct{984};
t50 = ct{985};
t500 = ct{986};
t501 = ct{987};
t502 = ct{988};
t503 = ct{989};
t504 = ct{990};
t505 = ct{991};
t506 = ct{992};
t507 = ct{993};
t508 = ct{994};
t509 = ct{995};
t51 = ct{996};
t510 = ct{997};
t511 = ct{998};
t514 = ct{999};
t515 = ct{1000};
t516 = ct{1001};
t519 = ct{1002};
t52 = ct{1003};
t520 = ct{1004};
t521 = ct{1005};
t522 = ct{1006};
t528 = ct{1007};
t53 = ct{1008};
t531 = ct{1009};
t532 = ct{1010};
t533 = ct{1011};
t537 = ct{1012};
t54 = ct{1013};
t545 = ct{1014};
t547 = ct{1015};
t548 = ct{1016};
t550 = ct{1017};
t553 = ct{1018};
t554 = ct{1019};
t555 = ct{1020};
t557 = ct{1021};
t559 = ct{1022};
t56 = ct{1023};
t560 = ct{1024};
t561 = ct{1025};
t562 = ct{1026};
t566 = ct{1027};
t568 = ct{1028};
t57 = ct{1029};
t570 = ct{1030};
t58 = ct{1031};
t582 = ct{1032};
t583 = ct{1033};
t584 = ct{1034};
t585 = ct{1035};
t589 = ct{1036};
t59 = ct{1037};
t590 = ct{1038};
t591 = ct{1039};
t592 = ct{1040};
t595 = ct{1041};
t597 = ct{1042};
t599 = ct{1043};
t6 = ct{1044};
t60 = ct{1045};
t600 = ct{1046};
t601 = ct{1047};
t605 = ct{1048};
t606 = ct{1049};
t607 = ct{1050};
t608 = ct{1051};
t609 = ct{1052};
t619 = ct{1053};
t620 = ct{1054};
t621 = ct{1055};
t622 = ct{1056};
t628 = ct{1057};
t63 = ct{1058};
t635 = ct{1059};
t636 = ct{1060};
t638 = ct{1061};
t64 = ct{1062};
t640 = ct{1063};
t641 = ct{1064};
t642 = ct{1065};
t643 = ct{1066};
t645 = ct{1067};
t646 = ct{1068};
t648 = ct{1069};
t649 = ct{1070};
t65 = ct{1071};
t654 = ct{1072};
t655 = ct{1073};
t656 = ct{1074};
t657 = ct{1075};
t659 = ct{1076};
t660 = ct{1077};
t663 = ct{1078};
t664 = ct{1079};
t665 = ct{1080};
t666 = ct{1081};
t667 = ct{1082};
t668 = ct{1083};
t669 = ct{1084};
t67 = ct{1085};
t670 = ct{1086};
t672 = ct{1087};
t673 = ct{1088};
t674 = ct{1089};
t675 = ct{1090};
t676 = ct{1091};
t677 = ct{1092};
t678 = ct{1093};
t679 = ct{1094};
t68 = ct{1095};
t681 = ct{1096};
t682 = ct{1097};
t683 = ct{1098};
t684 = ct{1099};
t685 = ct{1100};
t686 = ct{1101};
t687 = ct{1102};
t689 = ct{1103};
t69 = ct{1104};
t691 = ct{1105};
t692 = ct{1106};
t693 = ct{1107};
t694 = ct{1108};
t7 = ct{1109};
t70 = ct{1110};
t702 = ct{1111};
t704 = ct{1112};
t705 = ct{1113};
t707 = ct{1114};
t708 = ct{1115};
t71 = ct{1116};
t710 = ct{1117};
t711 = ct{1118};
t712 = ct{1119};
t713 = ct{1120};
t714 = ct{1121};
t715 = ct{1122};
t716 = ct{1123};
t717 = ct{1124};
t718 = ct{1125};
t719 = ct{1126};
t72 = ct{1127};
t720 = ct{1128};
t721 = ct{1129};
t722 = ct{1130};
t723 = ct{1131};
t724 = ct{1132};
t725 = ct{1133};
t726 = ct{1134};
t728 = ct{1135};
t73 = ct{1136};
t736 = ct{1137};
t738 = ct{1138};
t740 = ct{1139};
t741 = ct{1140};
t742 = ct{1141};
t743 = ct{1142};
t744 = ct{1143};
t745 = ct{1144};
t746 = ct{1145};
t747 = ct{1146};
t749 = ct{1147};
t75 = ct{1148};
t750 = ct{1149};
t751 = ct{1150};
t755 = ct{1151};
t756 = ct{1152};
t757 = ct{1153};
t758 = ct{1154};
t759 = ct{1155};
t76 = ct{1156};
t762 = ct{1157};
t763 = ct{1158};
t764 = ct{1159};
t766 = ct{1160};
t768 = ct{1161};
t77 = ct{1162};
t770 = ct{1163};
t771 = ct{1164};
t772 = ct{1165};
t773 = ct{1166};
t774 = ct{1167};
t775 = ct{1168};
t776 = ct{1169};
t777 = ct{1170};
t778 = ct{1171};
t78 = ct{1172};
t781 = ct{1173};
t782 = ct{1174};
t783 = ct{1175};
t784 = ct{1176};
t785 = ct{1177};
t786 = ct{1178};
t787 = ct{1179};
t789 = ct{1180};
t79 = ct{1181};
t790 = ct{1182};
t791 = ct{1183};
t792 = ct{1184};
t793 = ct{1185};
t794 = ct{1186};
t796 = ct{1187};
t797 = ct{1188};
t798 = ct{1189};
t799 = ct{1190};
t80 = ct{1191};
t800 = ct{1192};
t801 = ct{1193};
t802 = ct{1194};
t806 = ct{1195};
t807 = ct{1196};
t808 = ct{1197};
t809 = ct{1198};
t81 = ct{1199};
t812 = ct{1200};
t813 = ct{1201};
t816 = ct{1202};
t817 = ct{1203};
t818 = ct{1204};
t819 = ct{1205};
t82 = ct{1206};
t820 = ct{1207};
t821 = ct{1208};
t822 = ct{1209};
t823 = ct{1210};
t824 = ct{1211};
t825 = ct{1212};
t826 = ct{1213};
t827 = ct{1214};
t828 = ct{1215};
t829 = ct{1216};
t830 = ct{1217};
t831 = ct{1218};
t832 = ct{1219};
t833 = ct{1220};
t836 = ct{1221};
t837 = ct{1222};
t838 = ct{1223};
t839 = ct{1224};
t84 = ct{1225};
t840 = ct{1226};
t841 = ct{1227};
t844 = ct{1228};
t845 = ct{1229};
t846 = ct{1230};
t85 = ct{1231};
t850 = ct{1232};
t851 = ct{1233};
t852 = ct{1234};
t853 = ct{1235};
t854 = ct{1236};
t855 = ct{1237};
t857 = ct{1238};
t86 = ct{1239};
t860 = ct{1240};
t861 = ct{1241};
t863 = ct{1242};
t864 = ct{1243};
t866 = ct{1244};
t867 = ct{1245};
t869 = ct{1246};
t874 = ct{1247};
t875 = ct{1248};
t876 = ct{1249};
t877 = ct{1250};
t878 = ct{1251};
t882 = ct{1252};
t883 = ct{1253};
t887 = ct{1254};
t889 = ct{1255};
t89 = ct{1256};
t890 = ct{1257};
t896 = ct{1258};
t897 = ct{1259};
t898 = ct{1260};
t90 = ct{1261};
t900 = ct{1262};
t901 = ct{1263};
t902 = ct{1264};
t903 = ct{1265};
t904 = ct{1266};
t905 = ct{1267};
t906 = ct{1268};
t908 = ct{1269};
t909 = ct{1270};
t91 = ct{1271};
t913 = ct{1272};
t92 = ct{1273};
t920 = ct{1274};
t921 = ct{1275};
t923 = ct{1276};
t924 = ct{1277};
t929 = ct{1278};
t93 = ct{1279};
t938 = ct{1280};
t939 = ct{1281};
t94 = ct{1282};
t946 = ct{1283};
t95 = ct{1284};
t952 = ct{1285};
t954 = ct{1286};
t956 = ct{1287};
t957 = ct{1288};
t96 = ct{1289};
t963 = ct{1290};
t964 = ct{1291};
t97 = ct{1292};
t972 = ct{1293};
t975 = ct{1294};
t977 = ct{1295};
t98 = ct{1296};
t983 = ct{1297};
t986 = ct{1298};
t988 = ct{1299};
t99 = ct{1300};
t996 = ct{1301};
t998 = ct{1302};
t2625 = t27.*t30.*t31.*t32.*t50.*t202.*1.294536862550567e-20;
t2626 = t24.*t31.*t32.*t50.*t202.*5.999580612847032e-21;
t2627 = t25.*t30.*t32.*t50.*t202.*5.999580612847032e-21;
t2628 = t26.*t30.*t31.*t50.*t202.*5.999580612847032e-21;
t2631 = t30.*t31.*t32.*t33.*t50.*t202.*1.294536862550567e-20;
t2632 = t26.*t30.*t31.*t50.*t202.*(-3.566935413776081e-21);
t2633 = t30.*t31.*t32.*t50.*t202.*5.999580612847032e-21;
t2635 = t30.*t31.*t32.*t50.*t202.*(-3.566935413776081e-21);
t2639 = t24.*t25.*t26.*t50.*t202.*6.715770285417749e-24;
t2640 = t24.*t25.*t32.*t50.*t202.*(-3.992732227073824e-24);
t2641 = t24.*t25.*t32.*t50.*t202.*6.715770285417749e-24;
t2642 = t24.*t26.*t31.*t50.*t202.*6.715770285417749e-24;
t2643 = t25.*t26.*t30.*t50.*t202.*6.715770285417749e-24;
t2645 = t24.*t31.*t32.*t50.*t202.*(-3.992732227073824e-24);
t2646 = t25.*t30.*t32.*t50.*t202.*(-3.992732227073824e-24);
t2647 = t26.*t30.*t31.*t50.*t202.*(-3.992732227073824e-24);
t2651 = t24.*t31.*t32.*t50.*t202.*6.715770285417749e-24;
t2652 = t25.*t30.*t32.*t50.*t202.*6.715770285417749e-24;
t2653 = t26.*t30.*t31.*t50.*t202.*6.715770285417749e-24;
t2656 = t30.*t31.*t32.*t50.*t202.*6.715770285417749e-24;
t2723 = t24.*t25.*t50.*t202.*5.091703513734173e-22;
t2724 = t24.*t31.*t50.*t202.*5.091703513734173e-22;
t2725 = t25.*t30.*t50.*t202.*5.091703513734173e-22;
t2726 = t30.*t31.*t50.*t202.*5.091703513734173e-22;
t2727 = t24.*t25.*t50.*t202.*8.564238525144865e-22;
t2728 = t24.*t31.*t50.*t202.*8.564238525144865e-22;
t2729 = t25.*t30.*t50.*t202.*8.564238525144865e-22;
t2730 = t30.*t31.*t50.*t202.*8.564238525144865e-22;
t2735 = t38.*t50.*t202.*2.682760897261168e-21;
t2736 = t39.*t50.*t202.*2.682760897261168e-21;
t2745 = t24.*t25.*t50.*t202.*2.073708701385059e-20;
t2748 = t24.*t31.*t50.*t202.*2.073708701385059e-20;
t2749 = t25.*t30.*t50.*t202.*2.073708701385059e-20;
t2750 = t30.*t31.*t50.*t202.*2.073708701385059e-20;
t2773 = t38.*t50.*t202.*5.478197787607436e-20;
t2774 = t39.*t50.*t202.*5.478197787607436e-20;
t2775 = t24.*t25.*t50.*t202.*5.17981854669388e-20;
t2777 = t24.*t31.*t50.*t202.*5.17981854669388e-20;
t2778 = t25.*t30.*t50.*t202.*5.17981854669388e-20;
t2779 = t24.*t25.*t50.*t202.*3.079561623286356e-20;
t2780 = t30.*t31.*t50.*t202.*5.17981854669388e-20;
t2781 = t24.*t25.*t50.*t202.*3.487975272406493e-20;
t2782 = t24.*t31.*t50.*t202.*3.079561623286356e-20;
t2783 = t25.*t30.*t50.*t202.*3.079561623286356e-20;
t2785 = t24.*t31.*t50.*t202.*3.487975272406493e-20;
t2786 = t25.*t30.*t50.*t202.*3.487975272406493e-20;
t2787 = t30.*t31.*t50.*t202.*3.079561623286356e-20;
t2788 = t30.*t31.*t50.*t202.*3.487975272406493e-20;
t2797 = t38.*t50.*t202.*3.912111626280478e-20;
t2800 = t39.*t50.*t202.*3.912111626280478e-20;
t2857 = t24.*t25.*t26.*t27.*t50.*t202.*3.933139165631123e-21;
t2858 = t24.*t26.*t27.*t31.*t50.*t202.*3.933139165631123e-21;
t2859 = t25.*t26.*t27.*t30.*t50.*t202.*3.933139165631123e-21;
t2860 = t26.*t27.*t30.*t31.*t50.*t202.*3.933139165631123e-21;
t2865 = t24.*t25.*t32.*t50.*t202.*1.822828392793495e-21;
t2867 = t24.*t31.*t32.*t50.*t202.*1.822828392793495e-21;
t2868 = t25.*t30.*t32.*t50.*t202.*1.822828392793495e-21;
t2872 = t30.*t31.*t32.*t50.*t202.*1.822828392793495e-21;
t2879 = t24.*t25.*t32.*t50.*t202.*3.065994927666357e-21;
t2883 = t24.*t31.*t32.*t50.*t202.*3.065994927666357e-21;
t2884 = t25.*t30.*t32.*t50.*t202.*3.065994927666357e-21;
t2886 = t30.*t31.*t32.*t50.*t202.*3.065994927666357e-21;
t2887 = t24.*t25.*t26.*t33.*t50.*t202.*1.793448789769173e-21;
t2890 = t24.*t25.*t26.*t50.*t202.*2.040425413990593e-24;
t2891 = t24.*t26.*t31.*t33.*t50.*t202.*1.793448789769173e-21;
t2892 = t25.*t26.*t30.*t33.*t50.*t202.*1.793448789769173e-21;
t2894 = t24.*t26.*t31.*t50.*t202.*2.040425413990593e-24;
t2895 = t25.*t26.*t30.*t50.*t202.*2.040425413990593e-24;
t2896 = t24.*t25.*t26.*t27.*t50.*t202.*6.615534835481934e-21;
t2898 = t26.*t30.*t31.*t33.*t50.*t202.*1.793448789769173e-21;
t2899 = t26.*t30.*t31.*t50.*t202.*2.040425413990593e-24;
t2900 = t24.*t26.*t27.*t31.*t50.*t202.*6.615534835481934e-21;
t2901 = t25.*t26.*t27.*t30.*t50.*t202.*6.615534835481934e-21;
t2903 = t26.*t27.*t30.*t31.*t50.*t202.*6.615534835481934e-21;
t2905 = t24.*t25.*t26.*t33.*t50.*t202.*3.016578474529275e-21;
t2906 = t24.*t26.*t31.*t33.*t50.*t202.*3.016578474529275e-21;
t2907 = t25.*t26.*t30.*t33.*t50.*t202.*3.016578474529275e-21;
t2908 = t26.*t30.*t31.*t33.*t50.*t202.*3.016578474529275e-21;
t2915 = t24.*t25.*t26.*t50.*t202.*3.431992827360689e-24;
t2917 = t24.*t26.*t31.*t50.*t202.*3.431992827360689e-24;
t2918 = t25.*t26.*t30.*t50.*t202.*3.431992827360689e-24;
t2919 = t26.*t30.*t31.*t50.*t202.*3.431992827360689e-24;
t2959 = t50.*t188.*t202.*2.657710136023448e-22;
t2960 = t50.*t189.*t201.*2.657710136023448e-22;
t2963 = t50.*t188.*t202.*1.563956524727017e-23;
t2964 = t50.*t189.*t201.*1.563956524727017e-23;
t2967 = t50.*t188.*t202.*2.551073618220038e-22;
t2968 = t50.*t189.*t201.*2.551073618220038e-22;
t49 = -t46;
t131 = t43+t44;
t140 = t45+t48;
t268 = -t252;
t291 = t265.^2;
t292 = t250-1.0;
t335 = t237./1.0e+8;
t336 = t238./1.0e+8;
t337 = -t325;
t351 = -t340;
t352 = -t342;
t354 = -t344;
t356 = -t345;
t361 = -t348;
t362 = -t350;
t380 = -t366;
t387 = -t374;
t429 = t72+t86;
t512 = t237.*5.110348748545983e-1;
t513 = t238.*5.110348748545983e-1;
t517 = t262.*5.110348748545983e-1;
t518 = t264.*5.110348748545983e-1;
t523 = t237.*5.84482e-3;
t524 = t238.*5.84482e-3;
t525 = t237.*9.840000000000001e-6;
t526 = t238.*9.840000000000001e-6;
t527 = t240.*3.064357668490995e+34;
t530 = t237.*6.48e-5;
t536 = t238.*6.48e-5;
t538 = t17.*t237.*1.247162e-2;
t539 = t17.*t238.*1.247162e-2;
t540 = t22.*t238.*1.247162e-2;
t542 = t262.*5.84482e-3;
t543 = t264.*5.84482e-3;
t544 = t53.*t240;
t546 = t54.*t240;
t551 = t22.*t237.*5.68686e-3;
t552 = t17.*t238.*5.68686e-3;
t556 = t22.*t238.*5.68686e-3;
t563 = t262.*6.48e-5;
t565 = t264.*6.48e-5;
t569 = t237.*3.24e-6;
t571 = t237.*5.78002e-3;
t572 = t238.*3.24e-6;
t573 = t238.*5.78002e-3;
t574 = t237.*7.83e-6;
t575 = t237.*6.47e-6;
t576 = t238.*7.83e-6;
t577 = t238.*6.47e-6;
t578 = t237.*6.2e-7;
t580 = t238.*6.2e-7;
t610 = t262.*6.47e-6;
t611 = t264.*6.47e-6;
t612 = t237.*5.110348748545983e-9;
t613 = t98.*t240;
t614 = t99.*t240;
t615 = t100.*t240;
t616 = t101.*t240;
t617 = t102.*t240;
t618 = t103.*t240;
t623 = t107.*t240;
t624 = t108.*t240;
t625 = t109.*t240;
t627 = t110.*t240;
t629 = t111.*t240;
t630 = t112.*t240;
t631 = t113.*t240;
t634 = t114.*t240;
t637 = t117.*t240;
t650 = t26.*t28.*t240.*-3.315051378778914e+33;
t651 = t26.*t33.*t240.*7.788445287802242e+33;
t652 = t27.*t32.*t240.*-1.990083581481952e+33;
t658 = t27.*t34.*t240.*-1.025883768304404e+34;
t662 = t32.*t34.*t240.*-6.099194893302011e+33;
t696 = t128.*t240;
t697 = t129.*t240;
t698 = t130.*t240;
t701 = t132.*t240;
t733 = t134.*t240;
t734 = t135.*t240;
t735 = t136.*t240;
t737 = t137.*t240;
t739 = t27.*t32.*t34.*t240.*-3.315051378778914e+33;
t765 = t27.*t28.*t32.*t240.*-6.099194893302011e+33;
t767 = t139.*t240;
t847 = t146.*t240;
t849 = t147.*t240;
t856 = t26.*t240.*-7.746286054220548e+49;
t858 = t32.*t240.*-7.746286054220548e+49;
t859 = -t850;
t865 = -t855;
t868 = t160.*t240;
t870 = t161.*t240;
t871 = t162.*t240;
t872 = t16.*t850;
t873 = t21.*t850;
t881 = t167.*t240;
t884 = t169.*t240;
t885 = t172.*t240;
t886 = t163.*t240;
t888 = t164.*t240;
t891 = t26.*t855;
t892 = t32.*t855;
t893 = t32.*t240.*-6.997781708721691e+52;
t894 = t26.*t33.*t240.*-7.290917220067534e+49;
t895 = t32.*t33.*t240.*-7.290917220067534e+49;
t907 = t26.*t33.*t240.*7.342112502577776e+52;
t911 = t203.*t240;
t912 = t204.*t240;
t914 = t205.*t240;
t915 = t208.*t240;
t916 = t195.*t240;
t917 = t196.*t240;
t918 = t197.*t240;
t926 = t216.*t240;
t927 = t217.*t240;
t928 = t220.*t240;
t930 = t223.*t240;
t931 = t224.*t240;
t932 = t225.*t240;
t933 = t226.*t240;
t934 = t227.*t240;
t935 = t26.*t27.*t28.*t240.*-5.84291401185902e+49;
t936 = t230.*t240;
t937 = t231.*t240;
t940 = t32.*t34.*t240.*-2.201616617347892e+53;
t942 = t27.*t50.*t240.*7.432538878058787e+17i;
t943 = t26.*t28.*t240.*-1.196628789628727e+53;
t944 = (t123.*t237)./9.007199254740992e+15;
t945 = (t123.*t238)./9.007199254740992e+15;
t947 = t201+t258;
t948 = t188+t252-1.0;
t950 = t237.*(t42-t43).*(-1.110223024625157e-16);
t951 = t238.*(t42-t43).*(-1.110223024625157e-16);
t959 = t240.*t259;
t960 = t240.*t260;
t961 = t240.*t261;
t962 = t240.*t263;
t965 = t32.*t33.*t50.*t240.*4.418873226179514e+17i;
t966 = t240.*t271;
t967 = t240.*t272;
t968 = t240.*t273;
t969 = t240.*t274;
t970 = t240.*t255;
t971 = t240.*t256;
t973 = t240.*t257;
t974 = (t238.*(t42-t43))./9.007199254740992e+15;
t976 = t22.*t938;
t978 = t240.*t277;
t979 = t240.*t279;
t980 = t240.*t280;
t981 = t240.*t281;
t982 = t240.*t283;
t984 = t240.*t286;
t985 = t26.*t27.*t50.*t240.*-4.323455642275676e+17i;
t987 = t240.*t276;
t989 = -t972;
t990 = t32.*t33.*t50.*t240.*-4.323455642275676e+17i;
t992 = t26.*t34.*t50.*t240.*-1.325049802940888e+18i;
t993 = t28.*t32.*t50.*t240.*-1.325049802940888e+18i;
t994 = t32.*t34.*t50.*t240.*-1.325049802940888e+18i;
t995 = t32.*t34.*t50.*t240.*-7.201947557068188e+17i;
t997 = t238.*5.028583168569248e-6;
t999 = t244+t258+1.0;
t1007 = t240.*t301;
t1009 = t240.*t302;
t1010 = t240.*t303;
t1011 = t240.*t304;
t1012 = t240.*t305;
t1013 = t240.*t306;
t1014 = t240.*t307;
t1015 = t237.*2.986906857247653e-3;
t1016 = t240.*t308;
t1017 = t238.*2.986906857247653e-3;
t1018 = -t1002;
t1020 = t237.*3.311505989057797e-5;
t1021 = t238.*3.311505989057797e-5;
t1023 = t262.*(t46-t47).*(-1.110223024625157e-16);
t1024 = t22.*t237.*2.906183788415621e-3;
t1025 = t17.*t238.*2.906183788415621e-3;
t1027 = t264.*(t46-t47).*(-1.110223024625157e-16);
t1028 = t22.*t238.*2.906183788415621e-3;
t1029 = t26.*t27.*t28.*t50.*t240.*-1.325049802940888e+18i;
t1031 = -t1008;
t1032 = t26.*t27.*t34.*t50.*t240.*-7.201947557068188e+17i;
t1038 = t17.*t237.*6.373432765934105e-3;
t1041 = t17.*t238.*6.373432765934105e-3;
t1042 = t22.*t238.*6.373432765934105e-3;
t1045 = (t264.*(t46-t47))./9.007199254740992e+15;
t1046 = t262.*2.986906857247653e-3;
t1048 = t237.*3.168416224098509e-7;
t1050 = -t1035;
t1051 = t262.*3.311505989057797e-5;
t1052 = t237.*4.001403070111505e-6;
t1056 = t238.*2.953791797357075e-3;
t1057 = t237.*3.306395640309251e-6;
t1059 = t238.*3.306395640309251e-6;
t1061 = -t1047;
t1062 = t237.*1.655752994528898e-6;
t1072 = t264.*3.306395640309251e-6;
t1073 = t14.*t15.*t17.*t238.*1.07201054193752e-2;
t1074 = t14.*t17.*t20.*t238.*1.07201054193752e-2;
t1075 = t15.*t17.*t19.*t238.*1.07201054193752e-2;
t1076 = t17.*t19.*t20.*t238.*1.07201054193752e-2;
t1090 = t14.*t20.*t22.*t238.*4.888197259476159e-3;
t1091 = t15.*t19.*t22.*t238.*4.888197259476159e-3;
t1094 = t28.*t32.*t240.*1.297387533374166e+34;
t1095 = t19.*t20.*t22.*t238.*4.888197259476159e-3;
t1098 = t27.*t262.*1.35652563578e-4;
t1099 = t27.*t264.*1.35652563578e-4;
t1100 = t33.*t264.*1.35652563578e-4;
t1102 = t14.*t15.*t237.*2.953791797357075e-3;
t1103 = t32.*t34.*t240.*2.386997519508773e+34;
t1106 = t14.*t20.*t237.*2.953791797357075e-3;
t1107 = t15.*t19.*t237.*2.953791797357075e-3;
t1109 = t17.*t19.*t20.*t238.*(-6.373432765934105e-3);
t1111 = t19.*t20.*t237.*2.953791797357075e-3;
t1116 = t14.*t15.*t22.*t238.*(-2.906183788415621e-3);
t1117 = t33.*t262.*6.1855407534e-5;
t1118 = t27.*t264.*6.1855407534e-5;
t1119 = t14.*t20.*t22.*t238.*(-2.906183788415621e-3);
t1120 = t15.*t19.*t22.*t238.*(-2.906183788415621e-3);
t1122 = t33.*t264.*6.1855407534e-5;
t1125 = t14.*t15.*t22.*t238.*4.888197259476159e-3;
t1129 = t262.*7.0373543e-8;
t1132 = t14.*t15.*t238.*5.561353061058431e-6;
t1135 = t264.*7.0373543e-8;
t1138 = t14.*t20.*t238.*5.561353061058431e-6;
t1139 = t15.*t19.*t238.*5.561353061058431e-6;
t1140 = t19.*t20.*t238.*5.561353061058431e-6;
t1141 = t262.*6.2868699538e-5;
t1142 = t264.*6.2868699538e-5;
t1144 = t14.*t15.*t237.*4.968273867075572e-3;
t1146 = t14.*t20.*t237.*4.968273867075572e-3;
t1147 = t15.*t19.*t237.*4.968273867075572e-3;
t1149 = t19.*t20.*t237.*4.968273867075572e-3;
t1165 = t19.*t20.*t238.*(-3.306395640309251e-6);
t1171 = t240.*t373;
t1174 = t240.*t376;
t1186 = t26.*t33.*t34.*t240.*1.297387533374166e+34;
t1187 = t27.*t50.*t240.*-1.746965228796509e+32i;
t1188 = t26.*t28.*t33.*t240.*2.386997519508773e+34;
t1191 = t240.*t381;
t1195 = t240.*t384;
t1206 = t240.*t397;
t1209 = t240.*t398;
t1213 = t26.*t50.*t240.*-4.394953650240249e+33i;
t1224 = t240.*t405;
t1226 = t240.*t411;
t1228 = t240.*t412;
t1239 = t240.*t421;
t1240 = t240.*t422;
t1241 = t240.*t423;
t1244 = t240.*t428;
t1245 = t27.*t32.*t50.*t240.*-1.03862462117543e+32i;
t1250 = t240.*t430;
t1251 = t32.*t33.*t50.*t240.*-1.03862462117543e+32i;
t1257 = t240.*t437;
t1258 = t240.*t438;
t1259 = t240.*t439;
t1260 = t240.*t441;
t1261 = t240.*t442;
t1262 = t26.*t33.*t50.*t240.*-4.136594366080324e+33i;
t1263 = t27.*t32.*t50.*t240.*-4.136594366080324e+33i;
t1264 = t240.*t444;
t1266 = t26.*t50.*t240.*-3.97028021545552e+36i;
t1268 = t32.*t50.*t240.*-3.97028021545552e+36i;
t1270 = t27.*t28.*t50.*t240.*-1.025883768304404e+34i;
t1271 = t27.*t34.*t50.*t240.*-5.575912001630188e+33i;
t1272 = t28.*t33.*t50.*t240.*-5.575912001630188e+33i;
t1281 = -t1269;
t1282 = t240.*t466;
t1283 = t240.*t469;
t1296 = t22.*t1265;
t1304 = t240.*t470;
t1310 = t240.*t460;
t1314 = t240.*t461;
t1325 = t240.*t462;
t1326 = t240.*t463;
t1330 = t27.*t32.*t34.*t50.*t240.*-3.315051378778914e+33i;
t1331 = t32.*t33.*t50.*t240.*1.595073594941899e+37i;
t1332 = t32.*t33.*t34.*t50.*t240.*-3.315051378778914e+33i;
t1353 = t240.*t487;
t1359 = t240.*t488;
t1364 = t240.*t489;
t1365 = t240.*t490;
t1372 = t32.*t240.*7.152220999552773e+52;
t1377 = t240.*t492;
t1381 = t240.*t473;
t1382 = t240.*t474;
t1383 = t240.*t475;
t1388 = t32.*t33.*t50.*t240.*-4.075691174875038e+36i;
t1390 = t240.*t479;
t1391 = t240.*t480;
t1401 = -t1327;
t1402 = -t1329;
t1403 = t324+t349;
t1418 = t27.*t28.*t32.*t50.*t240.*-6.099194893302011e+33i;
t1422 = t27.*t32.*t34.*t50.*t240.*-6.099194893302011e+33i;
t1423 = t28.*t32.*t33.*t50.*t240.*-6.099194893302011e+33i;
t1426 = -t1373;
t1431 = t26.*t34.*t50.*t240.*-1.249115114148252e+37i;
t1432 = t28.*t32.*t50.*t240.*-1.249115114148252e+37i;
t1437 = t32.*t34.*t50.*t240.*-1.249115114148252e+37i;
t1439 = t32.*t34.*t50.*t240.*-6.789225223739216e+36i;
t1444 = t33.*t240.*3.147052781374869e+48;
t1449 = t240.*t503;
t1450 = t240.*t504;
t1451 = t240.*t505;
t1452 = t240.*t506;
t1453 = t32.*t34.*t240.*2.250205745048369e+53;
t1457 = t26.*t240.*7.917244648613035e+49;
t1459 = t28.*t32.*t240.*1.223038087510652e+53;
t1460 = t240.*t499;
t1461 = t240.*t500;
t1462 = t27.*t240.*1.253396129822139e+50;
t1463 = t240.*t501;
t1464 = t240.*t502;
t1468 = t27.*t32.*t240.*1.871019782761396e+48;
t1469 = -t1455;
t1471 = -t1456;
t1479 = -t1470;
t1482 = -t1473;
t1484 = -t1475;
t1485 = -t1477;
t1486 = t26.*t28.*t33.*t240.*2.250205745048369e+53;
t1487 = t33.*t34.*t240.*1.004467008511696e+50;
t1489 = t32.*t33.*t240.*7.451825938264896e+49;
t1494 = -t1481;
t1495 = t28.*t33.*t240.*1.848067902664462e+50;
t1499 = t26.*t33.*t34.*t240.*1.223038087510652e+53;
t1504 = -t1488;
t1505 = -t1493;
t1506 = -t1496;
t1507 = -t1498;
t1510 = t50.*t240.*6.804240878490729e+18i;
t1512 = -t1501;
t1516 = -t1503;
t1522 = -t1511;
t1525 = t27.*t28.*t32.*t240.*1.098733273949399e+50;
t1526 = -t1513;
t1527 = -t1515;
t1529 = -t1519;
t1531 = -t1521;
t1532 = t27.*t32.*t34.*t240.*5.971865661673106e+49;
t1533 = -t1524;
t1535 = t57+t58+t59+t95;
t1536 = t56+t73+t410;
t1543 = -t1537;
t1544 = t123.*t238.*6.489053738789607e-19;
t1547 = t123.*t238.*7.194245199571015e-21;
t1549 = t238.*(t42-t43).*(-6.489053738789607e-19);
t1550 = -t1545;
t1551 = t26.*t34.*t50.*t240.*1.354293320444013e+18i;
t1552 = t26.*t28.*t50.*t240.*7.360892737071442e+17i;
t1554 = t238.*(t42-t43).*(-7.194245199571015e-21);
t1555 = t27.*t28.*t50.*t240.*2.277919560321538e+18i;
t1556 = t27.*t34.*t50.*t240.*1.238101177498716e+18i;
t1558 = t238.*(t42-t43).*7.194245199571015e-21;
t1559 = t123.*t237.*7.183142969324763e-22;
t1565 = t237.*(t42-t43).*(-7.183142969324763e-22);
t1568 = -t1561;
t1569 = -t1562;
t1572 = -t1563;
t1574 = t28.*t32.*t33.*t50.*t240.*1.354293320444013e+18i;
t1575 = t32.*t33.*t34.*t50.*t240.*7.360892737071442e+17i;
t1579 = -t1566;
t1583 = -t1573;
t1588 = t22.*t237.*5.68686e-3;
t1592 = t17.*t237.*1.247162e-2;
t1594 = t238.*6.48e-5;
t1595 = -t1577;
t1596 = -t1578;
t1599 = t264.*(t46-t47).*(-6.489053738789607e-19);
t1600 = -t1581;
t1601 = -t1586;
t1602 = -t1587;
t1604 = -t1589;
t1605 = -t1590;
t1606 = -t1591;
t1613 = t264.*(t46-t47).*(-7.194245199571015e-21);
t1618 = t262.*3.601891949238275e-7;
t1619 = t264.*3.601891949238275e-7;
t1620 = t262.*8.631097478604537e-5;
t1622 = t264.*8.631097478604537e-5;
t1626 = -t1608;
t1627 = -t1609;
t1628 = -t1611;
t1629 = t19.*t20.*t238.*1.509490621508912e-3;
t1631 = -t1617;
t1633 = t14.*t15.*t17.*t237.*2.498039274760989e-3;
t1634 = t14.*t15.*t22.*t237.*2.498039274760989e-3;
t1635 = t14.*t17.*t20.*t237.*2.498039274760989e-3;
t1636 = t15.*t17.*t19.*t237.*2.498039274760989e-3;
t1637 = t14.*t15.*t17.*t237.*3.257046415933332e-3;
t1639 = t14.*t15.*t22.*t238.*2.498039274760989e-3;
t1640 = t14.*t20.*t22.*t237.*2.498039274760989e-3;
t1641 = t15.*t19.*t22.*t237.*2.498039274760989e-3;
t1642 = t17.*t19.*t20.*t237.*2.498039274760989e-3;
t1643 = t14.*t15.*t22.*t237.*3.257046415933332e-3;
t1644 = t14.*t15.*t17.*t238.*3.257046415933332e-3;
t1645 = t14.*t17.*t20.*t237.*3.257046415933332e-3;
t1646 = t15.*t17.*t19.*t237.*3.257046415933332e-3;
t1650 = t14.*t15.*t17.*t237.*1.485161268617439e-3;
t1651 = t14.*t15.*t17.*t237.*5.478347731418506e-3;
t1652 = t14.*t20.*t22.*t238.*2.498039274760989e-3;
t1653 = t15.*t19.*t22.*t238.*2.498039274760989e-3;
t1654 = t19.*t20.*t22.*t237.*2.498039274760989e-3;
t1655 = t14.*t20.*t22.*t237.*3.257046415933332e-3;
t1656 = t14.*t17.*t20.*t238.*3.257046415933332e-3;
t1657 = t15.*t19.*t22.*t237.*3.257046415933332e-3;
t1658 = t15.*t17.*t19.*t238.*3.257046415933332e-3;
